simulink model "model"  (R2016a)
(part 2 of 3)

  _CN_201293312_500000_CN_216778426_500000 : powerlib/Elements/Distributed Parameters Line  Phases=3  Frequency=50  Resistance=[0.01273 0.3864]  Inductance="[0.9337e-3  4.1264e-3]"  Capacitance=[12.74e-9 7.751e-9]  Length=28.6125  x1=[8.73114913702011e-11 380000 380000;314.159265358979 314.159265358979 314.159265358979;-0.177670123217348 0.415246442777429 -1.15554988401747]  x2=[1.26090477118469e-09 381852.398472139 381852.398472139;314.159265358979 314.159265358979 314.159265358979;-1.41941675517191 0.415007521738739 -1.15578880505616]  x3=[1.07663708898761e-11 1405.24743813465 1405.24743813466;314.159265358979 314.159265358979 314.159265358979;-2.70558821102223 0.316110507002444 -1.25468581979246]  x4=[8.62234243168895e-12 1405.96374414071 1405.9637441407;314.159265358979 314.159265358979 314.159265358979;0.245769282942371 0.405640215255436 -1.16515611153945]  x5=0.000565541566995742  V1=ones(3,3)  V2=ones(3,3)  I1=ones(3,3)  I2=ones(3,3)  nHarmo=1  Measurements=None
  _CN_215451416_500000_CN215429864 : powerlib/Elements/Distributed Parameters Line  Phases=3  Frequency=50  Resistance=[0.01273 0.3864]  Inductance="[0.9337e-3  4.1264e-3]"  Capacitance=[12.74e-9 7.751e-9]  Length=72.2446  x1=[8.73114913702011e-11 380000 380000;314.159265358979 314.159265358979 314.159265358979;-0.177670123217348 0.415246442777429 -1.15554988401747]  x2=[1.26090477118469e-09 381852.398472139 381852.398472139;314.159265358979 314.159265358979 314.159265358979;-1.41941675517191 0.415007521738739 -1.15578880505616]  x3=[1.07663708898761e-11 1405.24743813465 1405.24743813466;314.159265358979 314.159265358979 314.159265358979;-2.70558821102223 0.316110507002444 -1.25468581979246]  x4=[8.62234243168895e-12 1405.96374414071 1405.9637441407;314.159265358979 314.159265358979 314.159265358979;0.245769282942371 0.405640215255436 -1.16515611153945]  x5=0.000565541566995742  V1=ones(3,3)  V2=ones(3,3)  I1=ones(3,3)  I2=ones(3,3)  nHarmo=1  Measurements=None
  _CN_232998815_275000_CN233174201 : powerlib/Elements/Distributed Parameters Line  Phases=3  Frequency=50  Resistance=[0.01273 0.3864]  Inductance="[0.9337e-3  4.1264e-3]"  Capacitance=[12.74e-9 7.751e-9]  Length=1.0529  x1=[8.73114913702011e-11 380000 380000;314.159265358979 314.159265358979 314.159265358979;-0.177670123217348 0.415246442777429 -1.15554988401747]  x2=[1.26090477118469e-09 381852.398472139 381852.398472139;314.159265358979 314.159265358979 314.159265358979;-1.41941675517191 0.415007521738739 -1.15578880505616]  x3=[1.07663708898761e-11 1405.24743813465 1405.24743813466;314.159265358979 314.159265358979 314.159265358979;-2.70558821102223 0.316110507002444 -1.25468581979246]  x4=[8.62234243168895e-12 1405.96374414071 1405.9637441407;314.159265358979 314.159265358979 314.159265358979;0.245769282942371 0.405640215255436 -1.16515611153945]  x5=0.000565541566995742  V1=ones(3,3)  V2=ones(3,3)  I1=ones(3,3)  I2=ones(3,3)  nHarmo=1  Measurements=None
  _CN_241828221_500000_CN_241822623_500000 : powerlib/Elements/Distributed Parameters Line  Phases=3  Frequency=50  Resistance=[0.01273 0.3864]  Inductance="[0.9337e-3  4.1264e-3]"  Capacitance=[12.74e-9 7.751e-9]  Length=76.1994  x1=[8.73114913702011e-11 380000 380000;314.159265358979 314.159265358979 314.159265358979;-0.177670123217348 0.415246442777429 -1.15554988401747]  x2=[1.26090477118469e-09 381852.398472139 381852.398472139;314.159265358979 314.159265358979 314.159265358979;-1.41941675517191 0.415007521738739 -1.15578880505616]  x3=[1.07663708898761e-11 1405.24743813465 1405.24743813466;314.159265358979 314.159265358979 314.159265358979;-2.70558821102223 0.316110507002444 -1.25468581979246]  x4=[8.62234243168895e-12 1405.96374414071 1405.9637441407;314.159265358979 314.159265358979 314.159265358979;0.245769282942371 0.405640215255436 -1.16515611153945]  x5=0.000565541566995742  V1=ones(3,3)  V2=ones(3,3)  I1=ones(3,3)  I2=ones(3,3)  nHarmo=1  Measurements=None
  _CN_241956440_275000_CN214992492 : powerlib/Elements/Distributed Parameters Line  Phases=3  Frequency=50  Resistance=[0.01273 0.3864]  Inductance="[0.9337e-3  4.1264e-3]"  Capacitance=[12.74e-9 7.751e-9]  Length=68.4368  x1=[8.73114913702011e-11 380000 380000;314.159265358979 314.159265358979 314.159265358979;-0.177670123217348 0.415246442777429 -1.15554988401747]  x2=[1.26090477118469e-09 381852.398472139 381852.398472139;314.159265358979 314.159265358979 314.159265358979;-1.41941675517191 0.415007521738739 -1.15578880505616]  x3=[1.07663708898761e-11 1405.24743813465 1405.24743813466;314.159265358979 314.159265358979 314.159265358979;-2.70558821102223 0.316110507002444 -1.25468581979246]  x4=[8.62234243168895e-12 1405.96374414071 1405.9637441407;314.159265358979 314.159265358979 314.159265358979;0.245769282942371 0.405640215255436 -1.16515611153945]  x5=0.000565541566995742  V1=ones(3,3)  V2=ones(3,3)  I1=ones(3,3)  I2=ones(3,3)  nHarmo=1  Measurements=None
  _CN_241956440_275000_CN_241923317_275000 : powerlib/Elements/Distributed Parameters Line  Phases=3  Frequency=50  Resistance=[0.01273 0.3864]  Inductance="[0.9337e-3  4.1264e-3]"  Capacitance=[12.74e-9 7.751e-9]  Length=27.3525  x1=[8.73114913702011e-11 380000 380000;314.159265358979 314.159265358979 314.159265358979;-0.177670123217348 0.415246442777429 -1.15554988401747]  x2=[1.26090477118469e-09 381852.398472139 381852.398472139;314.159265358979 314.159265358979 314.159265358979;-1.41941675517191 0.415007521738739 -1.15578880505616]  x3=[1.07663708898761e-11 1405.24743813465 1405.24743813466;314.159265358979 314.159265358979 314.159265358979;-2.70558821102223 0.316110507002444 -1.25468581979246]  x4=[8.62234243168895e-12 1405.96374414071 1405.9637441407;314.159265358979 314.159265358979 314.159265358979;0.245769282942371 0.405640215255436 -1.16515611153945]  x5=0.000565541566995742  V1=ones(3,3)  V2=ones(3,3)  I1=ones(3,3)  I2=ones(3,3)  nHarmo=1  Measurements=None
  _CN_241956440_275000_CN_242532736_275000 : powerlib/Elements/Distributed Parameters Line  Phases=3  Frequency=50  Resistance=[0.01273 0.3864]  Inductance="[0.9337e-3  4.1264e-3]"  Capacitance=[12.74e-9 7.751e-9]  Length=38.0576  x1=[8.73114913702011e-11 380000 380000;314.159265358979 314.159265358979 314.159265358979;-0.177670123217348 0.415246442777429 -1.15554988401747]  x2=[1.26090477118469e-09 381852.398472139 381852.398472139;314.159265358979 314.159265358979 314.159265358979;-1.41941675517191 0.415007521738739 -1.15578880505616]  x3=[1.07663708898761e-11 1405.24743813465 1405.24743813466;314.159265358979 314.159265358979 314.159265358979;-2.70558821102223 0.316110507002444 -1.25468581979246]  x4=[8.62234243168895e-12 1405.96374414071 1405.9637441407;314.159265358979 314.159265358979 314.159265358979;0.245769282942371 0.405640215255436 -1.16515611153945]  x5=0.000565541566995742  V1=ones(3,3)  V2=ones(3,3)  I1=ones(3,3)  I2=ones(3,3)  nHarmo=1  Measurements=None
  _CN_242103481_500000_CN_241828221_500000 : powerlib/Elements/Distributed Parameters Line  Phases=3  Frequency=50  Resistance=[0.01273 0.3864]  Inductance="[0.9337e-3  4.1264e-3]"  Capacitance=[12.74e-9 7.751e-9]  Length=71.051  x1=[8.73114913702011e-11 380000 380000;314.159265358979 314.159265358979 314.159265358979;-0.177670123217348 0.415246442777429 -1.15554988401747]  x2=[1.26090477118469e-09 381852.398472139 381852.398472139;314.159265358979 314.159265358979 314.159265358979;-1.41941675517191 0.415007521738739 -1.15578880505616]  x3=[1.07663708898761e-11 1405.24743813465 1405.24743813466;314.159265358979 314.159265358979 314.159265358979;-2.70558821102223 0.316110507002444 -1.25468581979246]  x4=[8.62234243168895e-12 1405.96374414071 1405.9637441407;314.159265358979 314.159265358979 314.159265358979;0.245769282942371 0.405640215255436 -1.16515611153945]  x5=0.000565541566995742  V1=ones(3,3)  V2=ones(3,3)  I1=ones(3,3)  I2=ones(3,3)  nHarmo=1  Measurements=None
  _CN_242103481_500000_CN_317416612_500000 : powerlib/Elements/Distributed Parameters Line  Phases=3  Frequency=50  Resistance=[0.01273 0.3864]  Inductance="[0.9337e-3  4.1264e-3]"  Capacitance=[12.74e-9 7.751e-9]  Length=86.3859  x1=[8.73114913702011e-11 380000 380000;314.159265358979 314.159265358979 314.159265358979;-0.177670123217348 0.415246442777429 -1.15554988401747]  x2=[1.26090477118469e-09 381852.398472139 381852.398472139;314.159265358979 314.159265358979 314.159265358979;-1.41941675517191 0.415007521738739 -1.15578880505616]  x3=[1.07663708898761e-11 1405.24743813465 1405.24743813466;314.159265358979 314.159265358979 314.159265358979;-2.70558821102223 0.316110507002444 -1.25468581979246]  x4=[8.62234243168895e-12 1405.96374414071 1405.9637441407;314.159265358979 314.159265358979 314.159265358979;0.245769282942371 0.405640215255436 -1.16515611153945]  x5=0.000565541566995742  V1=ones(3,3)  V2=ones(3,3)  I1=ones(3,3)  I2=ones(3,3)  nHarmo=1  Measurements=None
  _CN_242103481_500000_CN_317511904_500000 : powerlib/Elements/Distributed Parameters Line  Phases=3  Frequency=50  Resistance=[0.01273 0.3864]  Inductance="[0.9337e-3  4.1264e-3]"  Capacitance=[12.74e-9 7.751e-9]  Length=50.2566  x1=[8.73114913702011e-11 380000 380000;314.159265358979 314.159265358979 314.159265358979;-0.177670123217348 0.415246442777429 -1.15554988401747]  x2=[1.26090477118469e-09 381852.398472139 381852.398472139;314.159265358979 314.159265358979 314.159265358979;-1.41941675517191 0.415007521738739 -1.15578880505616]  x3=[1.07663708898761e-11 1405.24743813465 1405.24743813466;314.159265358979 314.159265358979 314.159265358979;-2.70558821102223 0.316110507002444 -1.25468581979246]  x4=[8.62234243168895e-12 1405.96374414071 1405.9637441407;314.159265358979 314.159265358979 314.159265358979;0.245769282942371 0.405640215255436 -1.16515611153945]  x5=0.000565541566995742  V1=ones(3,3)  V2=ones(3,3)  I1=ones(3,3)  I2=ones(3,3)  nHarmo=1  Measurements=None
  _CN_242103532_500000_CN_241822623_500000 : powerlib/Elements/Distributed Parameters Line  Phases=3  Frequency=50  Resistance=[0.01273 0.3864]  Inductance="[0.9337e-3  4.1264e-3]"  Capacitance=[12.74e-9 7.751e-9]  Length=4.2886  x1=[8.73114913702011e-11 380000 380000;314.159265358979 314.159265358979 314.159265358979;-0.177670123217348 0.415246442777429 -1.15554988401747]  x2=[1.26090477118469e-09 381852.398472139 381852.398472139;314.159265358979 314.159265358979 314.159265358979;-1.41941675517191 0.415007521738739 -1.15578880505616]  x3=[1.07663708898761e-11 1405.24743813465 1405.24743813466;314.159265358979 314.159265358979 314.159265358979;-2.70558821102223 0.316110507002444 -1.25468581979246]  x4=[8.62234243168895e-12 1405.96374414071 1405.9637441407;314.159265358979 314.159265358979 314.159265358979;0.245769282942371 0.405640215255436 -1.16515611153945]  x5=0.000565541566995742  V1=ones(3,3)  V2=ones(3,3)  I1=ones(3,3)  I2=ones(3,3)  nHarmo=1  Measurements=None
  _CN_242253497_275000_CN_185032690_275000 : powerlib/Elements/Distributed Parameters Line  Phases=3  Frequency=50  Resistance=[0.01273 0.3864]  Inductance="[0.9337e-3  4.1264e-3]"  Capacitance=[12.74e-9 7.751e-9]  Length=66.6304  x1=[8.73114913702011e-11 380000 380000;314.159265358979 314.159265358979 314.159265358979;-0.177670123217348 0.415246442777429 -1.15554988401747]  x2=[1.26090477118469e-09 381852.398472139 381852.398472139;314.159265358979 314.159265358979 314.159265358979;-1.41941675517191 0.415007521738739 -1.15578880505616]  x3=[1.07663708898761e-11 1405.24743813465 1405.24743813466;314.159265358979 314.159265358979 314.159265358979;-2.70558821102223 0.316110507002444 -1.25468581979246]  x4=[8.62234243168895e-12 1405.96374414071 1405.9637441407;314.159265358979 314.159265358979 314.159265358979;0.245769282942371 0.405640215255436 -1.16515611153945]  x5=0.000565541566995742  V1=ones(3,3)  V2=ones(3,3)  I1=ones(3,3)  I2=ones(3,3)  nHarmo=1  Measurements=None
  _CN_242253500_500000_CN_204258596_500000 : powerlib/Elements/Distributed Parameters Line  Phases=3  Frequency=50  Resistance=[0.01273 0.3864]  Inductance="[0.9337e-3  4.1264e-3]"  Capacitance=[12.74e-9 7.751e-9]  Length=93.4711  x1=[8.73114913702011e-11 380000 380000;314.159265358979 314.159265358979 314.159265358979;-0.177670123217348 0.415246442777429 -1.15554988401747]  x2=[1.26090477118469e-09 381852.398472139 381852.398472139;314.159265358979 314.159265358979 314.159265358979;-1.41941675517191 0.415007521738739 -1.15578880505616]  x3=[1.07663708898761e-11 1405.24743813465 1405.24743813466;314.159265358979 314.159265358979 314.159265358979;-2.70558821102223 0.316110507002444 -1.25468581979246]  x4=[8.62234243168895e-12 1405.96374414071 1405.9637441407;314.159265358979 314.159265358979 314.159265358979;0.245769282942371 0.405640215255436 -1.16515611153945]  x5=0.000565541566995742  V1=ones(3,3)  V2=ones(3,3)  I1=ones(3,3)  I2=ones(3,3)  nHarmo=1  Measurements=None
  _CN_250430935_275000_CN354115662 : powerlib/Elements/Distributed Parameters Line  Phases=3  Frequency=50  Resistance=[0.01273 0.3864]  Inductance="[0.9337e-3  4.1264e-3]"  Capacitance=[12.74e-9 7.751e-9]  Length=98.2855  x1=[8.73114913702011e-11 380000 380000;314.159265358979 314.159265358979 314.159265358979;-0.177670123217348 0.415246442777429 -1.15554988401747]  x2=[1.26090477118469e-09 381852.398472139 381852.398472139;314.159265358979 314.159265358979 314.159265358979;-1.41941675517191 0.415007521738739 -1.15578880505616]  x3=[1.07663708898761e-11 1405.24743813465 1405.24743813466;314.159265358979 314.159265358979 314.159265358979;-2.70558821102223 0.316110507002444 -1.25468581979246]  x4=[8.62234243168895e-12 1405.96374414071 1405.9637441407;314.159265358979 314.159265358979 314.159265358979;0.245769282942371 0.405640215255436 -1.16515611153945]  x5=0.000565541566995742  V1=ones(3,3)  V2=ones(3,3)  I1=ones(3,3)  I2=ones(3,3)  nHarmo=1  Measurements=None
  _CN_250430935_275000_CN_107262429_275000 : powerlib/Elements/Distributed Parameters Line  Phases=3  Frequency=50  Resistance=[0.01273 0.3864]  Inductance="[0.9337e-3  4.1264e-3]"  Capacitance=[12.74e-9 7.751e-9]  Length=49.0738  x1=[8.73114913702011e-11 380000 380000;314.159265358979 314.159265358979 314.159265358979;-0.177670123217348 0.415246442777429 -1.15554988401747]  x2=[1.26090477118469e-09 381852.398472139 381852.398472139;314.159265358979 314.159265358979 314.159265358979;-1.41941675517191 0.415007521738739 -1.15578880505616]  x3=[1.07663708898761e-11 1405.24743813465 1405.24743813466;314.159265358979 314.159265358979 314.159265358979;-2.70558821102223 0.316110507002444 -1.25468581979246]  x4=[8.62234243168895e-12 1405.96374414071 1405.9637441407;314.159265358979 314.159265358979 314.159265358979;0.245769282942371 0.405640215255436 -1.16515611153945]  x5=0.000565541566995742  V1=ones(3,3)  V2=ones(3,3)  I1=ones(3,3)  I2=ones(3,3)  nHarmo=1  Measurements=None
  _CN_302164679_275000_CN_316581637_275000 : powerlib/Elements/Distributed Parameters Line  Phases=3  Frequency=50  Resistance=[0.01273 0.3864]  Inductance="[0.9337e-3  4.1264e-3]"  Capacitance=[12.74e-9 7.751e-9]  Length=35.2995  x1=[8.73114913702011e-11 380000 380000;314.159265358979 314.159265358979 314.159265358979;-0.177670123217348 0.415246442777429 -1.15554988401747]  x2=[1.26090477118469e-09 381852.398472139 381852.398472139;314.159265358979 314.159265358979 314.159265358979;-1.41941675517191 0.415007521738739 -1.15578880505616]  x3=[1.07663708898761e-11 1405.24743813465 1405.24743813466;314.159265358979 314.159265358979 314.159265358979;-2.70558821102223 0.316110507002444 -1.25468581979246]  x4=[8.62234243168895e-12 1405.96374414071 1405.9637441407;314.159265358979 314.159265358979 314.159265358979;0.245769282942371 0.405640215255436 -1.16515611153945]  x5=0.000565541566995742  V1=ones(3,3)  V2=ones(3,3)  I1=ones(3,3)  I2=ones(3,3)  nHarmo=1  Measurements=None
  _CN_315461272_500000_CN_105298089_500000 : powerlib/Elements/Distributed Parameters Line  Phases=3  Frequency=50  Resistance=[0.01273 0.3864]  Inductance="[0.9337e-3  4.1264e-3]"  Capacitance=[12.74e-9 7.751e-9]  Length=97.8057  x1=[8.73114913702011e-11 380000 380000;314.159265358979 314.159265358979 314.159265358979;-0.177670123217348 0.415246442777429 -1.15554988401747]  x2=[1.26090477118469e-09 381852.398472139 381852.398472139;314.159265358979 314.159265358979 314.159265358979;-1.41941675517191 0.415007521738739 -1.15578880505616]  x3=[1.07663708898761e-11 1405.24743813465 1405.24743813466;314.159265358979 314.159265358979 314.159265358979;-2.70558821102223 0.316110507002444 -1.25468581979246]  x4=[8.62234243168895e-12 1405.96374414071 1405.9637441407;314.159265358979 314.159265358979 314.159265358979;0.245769282942371 0.405640215255436 -1.16515611153945]  x5=0.000565541566995742  V1=ones(3,3)  V2=ones(3,3)  I1=ones(3,3)  I2=ones(3,3)  nHarmo=1  Measurements=None
  _CN_315608215_500000_CN_169249243_500000 : powerlib/Elements/Distributed Parameters Line  Phases=3  Frequency=50  Resistance=[0.01273 0.3864]  Inductance="[0.9337e-3  4.1264e-3]"  Capacitance=[12.74e-9 7.751e-9]  Length=85.9807  x1=[8.73114913702011e-11 380000 380000;314.159265358979 314.159265358979 314.159265358979;-0.177670123217348 0.415246442777429 -1.15554988401747]  x2=[1.26090477118469e-09 381852.398472139 381852.398472139;314.159265358979 314.159265358979 314.159265358979;-1.41941675517191 0.415007521738739 -1.15578880505616]  x3=[1.07663708898761e-11 1405.24743813465 1405.24743813466;314.159265358979 314.159265358979 314.159265358979;-2.70558821102223 0.316110507002444 -1.25468581979246]  x4=[8.62234243168895e-12 1405.96374414071 1405.9637441407;314.159265358979 314.159265358979 314.159265358979;0.245769282942371 0.405640215255436 -1.16515611153945]  x5=0.000565541566995742  V1=ones(3,3)  V2=ones(3,3)  I1=ones(3,3)  I2=ones(3,3)  nHarmo=1  Measurements=None
  _CN_315608215_500000_CN_169249247_500000 : powerlib/Elements/Distributed Parameters Line  Phases=3  Frequency=50  Resistance=[0.01273 0.3864]  Inductance="[0.9337e-3  4.1264e-3]"  Capacitance=[12.74e-9 7.751e-9]  Length=76.4137  x1=[8.73114913702011e-11 380000 380000;314.159265358979 314.159265358979 314.159265358979;-0.177670123217348 0.415246442777429 -1.15554988401747]  x2=[1.26090477118469e-09 381852.398472139 381852.398472139;314.159265358979 314.159265358979 314.159265358979;-1.41941675517191 0.415007521738739 -1.15578880505616]  x3=[1.07663708898761e-11 1405.24743813465 1405.24743813466;314.159265358979 314.159265358979 314.159265358979;-2.70558821102223 0.316110507002444 -1.25468581979246]  x4=[8.62234243168895e-12 1405.96374414071 1405.9637441407;314.159265358979 314.159265358979 314.159265358979;0.245769282942371 0.405640215255436 -1.16515611153945]  x5=0.000565541566995742  V1=ones(3,3)  V2=ones(3,3)  I1=ones(3,3)  I2=ones(3,3)  nHarmo=1  Measurements=None
  _CN_315614776_275000_CN_315614783_275000 : powerlib/Elements/Distributed Parameters Line  Phases=3  Frequency=50  Resistance=[0.01273 0.3864]  Inductance="[0.9337e-3  4.1264e-3]"  Capacitance=[12.74e-9 7.751e-9]  Length=12.0528  x1=[8.73114913702011e-11 380000 380000;314.159265358979 314.159265358979 314.159265358979;-0.177670123217348 0.415246442777429 -1.15554988401747]  x2=[1.26090477118469e-09 381852.398472139 381852.398472139;314.159265358979 314.159265358979 314.159265358979;-1.41941675517191 0.415007521738739 -1.15578880505616]  x3=[1.07663708898761e-11 1405.24743813465 1405.24743813466;314.159265358979 314.159265358979 314.159265358979;-2.70558821102223 0.316110507002444 -1.25468581979246]  x4=[8.62234243168895e-12 1405.96374414071 1405.9637441407;314.159265358979 314.159265358979 314.159265358979;0.245769282942371 0.405640215255436 -1.16515611153945]  x5=0.000565541566995742  V1=ones(3,3)  V2=ones(3,3)  I1=ones(3,3)  I2=ones(3,3)  nHarmo=1  Measurements=None
  _CN_316459359_275000_CN_107262429_275000 : powerlib/Elements/Distributed Parameters Line  Phases=3  Frequency=50  Resistance=[0.01273 0.3864]  Inductance="[0.9337e-3  4.1264e-3]"  Capacitance=[12.74e-9 7.751e-9]  Length=29.441  x1=[8.73114913702011e-11 380000 380000;314.159265358979 314.159265358979 314.159265358979;-0.177670123217348 0.415246442777429 -1.15554988401747]  x2=[1.26090477118469e-09 381852.398472139 381852.398472139;314.159265358979 314.159265358979 314.159265358979;-1.41941675517191 0.415007521738739 -1.15578880505616]  x3=[1.07663708898761e-11 1405.24743813465 1405.24743813466;314.159265358979 314.159265358979 314.159265358979;-2.70558821102223 0.316110507002444 -1.25468581979246]  x4=[8.62234243168895e-12 1405.96374414071 1405.9637441407;314.159265358979 314.159265358979 314.159265358979;0.245769282942371 0.405640215255436 -1.16515611153945]  x5=0.000565541566995742  V1=ones(3,3)  V2=ones(3,3)  I1=ones(3,3)  I2=ones(3,3)  nHarmo=1  Measurements=None
  _CN_316566585_275000_CN_174636874_275000 : powerlib/Elements/Distributed Parameters Line  Phases=3  Frequency=50  Resistance=[0.01273 0.3864]  Inductance="[0.9337e-3  4.1264e-3]"  Capacitance=[12.74e-9 7.751e-9]  Length=36.4336  x1=[8.73114913702011e-11 380000 380000;314.159265358979 314.159265358979 314.159265358979;-0.177670123217348 0.415246442777429 -1.15554988401747]  x2=[1.26090477118469e-09 381852.398472139 381852.398472139;314.159265358979 314.159265358979 314.159265358979;-1.41941675517191 0.415007521738739 -1.15578880505616]  x3=[1.07663708898761e-11 1405.24743813465 1405.24743813466;314.159265358979 314.159265358979 314.159265358979;-2.70558821102223 0.316110507002444 -1.25468581979246]  x4=[8.62234243168895e-12 1405.96374414071 1405.9637441407;314.159265358979 314.159265358979 314.159265358979;0.245769282942371 0.405640215255436 -1.16515611153945]  x5=0.000565541566995742  V1=ones(3,3)  V2=ones(3,3)  I1=ones(3,3)  I2=ones(3,3)  nHarmo=1  Measurements=None
  _CN_316566588_275000_CN_174636874_275000 : powerlib/Elements/Distributed Parameters Line  Phases=3  Frequency=50  Resistance=[0.01273 0.3864]  Inductance="[0.9337e-3  4.1264e-3]"  Capacitance=[12.74e-9 7.751e-9]  Length=100.2417  x1=[8.73114913702011e-11 380000 380000;314.159265358979 314.159265358979 314.159265358979;-0.177670123217348 0.415246442777429 -1.15554988401747]  x2=[1.26090477118469e-09 381852.398472139 381852.398472139;314.159265358979 314.159265358979 314.159265358979;-1.41941675517191 0.415007521738739 -1.15578880505616]  x3=[1.07663708898761e-11 1405.24743813465 1405.24743813466;314.159265358979 314.159265358979 314.159265358979;-2.70558821102223 0.316110507002444 -1.25468581979246]  x4=[8.62234243168895e-12 1405.96374414071 1405.9637441407;314.159265358979 314.159265358979 314.159265358979;0.245769282942371 0.405640215255436 -1.16515611153945]  x5=0.000565541566995742  V1=ones(3,3)  V2=ones(3,3)  I1=ones(3,3)  I2=ones(3,3)  nHarmo=1  Measurements=None
  _CN_316566588_275000_CN_308348224_275000 : powerlib/Elements/Distributed Parameters Line  Phases=3  Frequency=50  Resistance=[0.01273 0.3864]  Inductance="[0.9337e-3  4.1264e-3]"  Capacitance=[12.74e-9 7.751e-9]  Length=168.728  x1=[8.73114913702011e-11 380000 380000;314.159265358979 314.159265358979 314.159265358979;-0.177670123217348 0.415246442777429 -1.15554988401747]  x2=[1.26090477118469e-09 381852.398472139 381852.398472139;314.159265358979 314.159265358979 314.159265358979;-1.41941675517191 0.415007521738739 -1.15578880505616]  x3=[1.07663708898761e-11 1405.24743813465 1405.24743813466;314.159265358979 314.159265358979 314.159265358979;-2.70558821102223 0.316110507002444 -1.25468581979246]  x4=[8.62234243168895e-12 1405.96374414071 1405.9637441407;314.159265358979 314.159265358979 314.159265358979;0.245769282942371 0.405640215255436 -1.16515611153945]  x5=0.000565541566995742  V1=ones(3,3)  V2=ones(3,3)  I1=ones(3,3)  I2=ones(3,3)  nHarmo=1  Measurements=None
  _CN_316566588_275000_CN_316581632_275000 : powerlib/Elements/Distributed Parameters Line  Phases=3  Frequency=50  Resistance=[0.01273 0.3864]  Inductance="[0.9337e-3  4.1264e-3]"  Capacitance=[12.74e-9 7.751e-9]  Length=2.0576  x1=[8.73114913702011e-11 380000 380000;314.159265358979 314.159265358979 314.159265358979;-0.177670123217348 0.415246442777429 -1.15554988401747]  x2=[1.26090477118469e-09 381852.398472139 381852.398472139;314.159265358979 314.159265358979 314.159265358979;-1.41941675517191 0.415007521738739 -1.15578880505616]  x3=[1.07663708898761e-11 1405.24743813465 1405.24743813466;314.159265358979 314.159265358979 314.159265358979;-2.70558821102223 0.316110507002444 -1.25468581979246]  x4=[8.62234243168895e-12 1405.96374414071 1405.9637441407;314.159265358979 314.159265358979 314.159265358979;0.245769282942371 0.405640215255436 -1.16515611153945]  x5=0.000565541566995742  V1=ones(3,3)  V2=ones(3,3)  I1=ones(3,3)  I2=ones(3,3)  nHarmo=1  Measurements=None
  _CN_317416612_500000_CN_204258596_500000 : powerlib/Elements/Distributed Parameters Line  Phases=3  Frequency=50  Resistance=[0.01273 0.3864]  Inductance="[0.9337e-3  4.1264e-3]"  Capacitance=[12.74e-9 7.751e-9]  Length=29.4625  x1=[8.73114913702011e-11 380000 380000;314.159265358979 314.159265358979 314.159265358979;-0.177670123217348 0.415246442777429 -1.15554988401747]  x2=[1.26090477118469e-09 381852.398472139 381852.398472139;314.159265358979 314.159265358979 314.159265358979;-1.41941675517191 0.415007521738739 -1.15578880505616]  x3=[1.07663708898761e-11 1405.24743813465 1405.24743813466;314.159265358979 314.159265358979 314.159265358979;-2.70558821102223 0.316110507002444 -1.25468581979246]  x4=[8.62234243168895e-12 1405.96374414071 1405.9637441407;314.159265358979 314.159265358979 314.159265358979;0.245769282942371 0.405640215255436 -1.16515611153945]  x5=0.000565541566995742  V1=ones(3,3)  V2=ones(3,3)  I1=ones(3,3)  I2=ones(3,3)  nHarmo=1  Measurements=None
  _CN_318218831_275000_CN_169993955_275000 : powerlib/Elements/Distributed Parameters Line  Phases=3  Frequency=50  Resistance=[0.01273 0.3864]  Inductance="[0.9337e-3  4.1264e-3]"  Capacitance=[12.74e-9 7.751e-9]  Length=37.4693  x1=[8.73114913702011e-11 380000 380000;314.159265358979 314.159265358979 314.159265358979;-0.177670123217348 0.415246442777429 -1.15554988401747]  x2=[1.26090477118469e-09 381852.398472139 381852.398472139;314.159265358979 314.159265358979 314.159265358979;-1.41941675517191 0.415007521738739 -1.15578880505616]  x3=[1.07663708898761e-11 1405.24743813465 1405.24743813466;314.159265358979 314.159265358979 314.159265358979;-2.70558821102223 0.316110507002444 -1.25468581979246]  x4=[8.62234243168895e-12 1405.96374414071 1405.9637441407;314.159265358979 314.159265358979 314.159265358979;0.245769282942371 0.405640215255436 -1.16515611153945]  x5=0.000565541566995742  V1=ones(3,3)  V2=ones(3,3)  I1=ones(3,3)  I2=ones(3,3)  nHarmo=1  Measurements=None
  _CN_318218831_275000_CN_170016148_275000 : powerlib/Elements/Distributed Parameters Line  Phases=3  Frequency=50  Resistance=[0.01273 0.3864]  Inductance="[0.9337e-3  4.1264e-3]"  Capacitance=[12.74e-9 7.751e-9]  Length=35.0104  x1=[8.73114913702011e-11 380000 380000;314.159265358979 314.159265358979 314.159265358979;-0.177670123217348 0.415246442777429 -1.15554988401747]  x2=[1.26090477118469e-09 381852.398472139 381852.398472139;314.159265358979 314.159265358979 314.159265358979;-1.41941675517191 0.415007521738739 -1.15578880505616]  x3=[1.07663708898761e-11 1405.24743813465 1405.24743813466;314.159265358979 314.159265358979 314.159265358979;-2.70558821102223 0.316110507002444 -1.25468581979246]  x4=[8.62234243168895e-12 1405.96374414071 1405.9637441407;314.159265358979 314.159265358979 314.159265358979;0.245769282942371 0.405640215255436 -1.16515611153945]  x5=0.000565541566995742  V1=ones(3,3)  V2=ones(3,3)  I1=ones(3,3)  I2=ones(3,3)  nHarmo=1  Measurements=None
  _CN_318218831_275000_CN_319300956_275000 : powerlib/Elements/Distributed Parameters Line  Phases=3  Frequency=50  Resistance=[0.01273 0.3864]  Inductance="[0.9337e-3  4.1264e-3]"  Capacitance=[12.74e-9 7.751e-9]  Length=85.9941  x1=[8.73114913702011e-11 380000 380000;314.159265358979 314.159265358979 314.159265358979;-0.177670123217348 0.415246442777429 -1.15554988401747]  x2=[1.26090477118469e-09 381852.398472139 381852.398472139;314.159265358979 314.159265358979 314.159265358979;-1.41941675517191 0.415007521738739 -1.15578880505616]  x3=[1.07663708898761e-11 1405.24743813465 1405.24743813466;314.159265358979 314.159265358979 314.159265358979;-2.70558821102223 0.316110507002444 -1.25468581979246]  x4=[8.62234243168895e-12 1405.96374414071 1405.9637441407;314.159265358979 314.159265358979 314.159265358979;0.245769282942371 0.405640215255436 -1.16515611153945]  x5=0.000565541566995742  V1=ones(3,3)  V2=ones(3,3)  I1=ones(3,3)  I2=ones(3,3)  nHarmo=1  Measurements=None
  _CN_318302348_275000_CN319098734 : powerlib/Elements/Distributed Parameters Line  Phases=3  Frequency=50  Resistance=[0.01273 0.3864]  Inductance="[0.9337e-3  4.1264e-3]"  Capacitance=[12.74e-9 7.751e-9]  Length=47.29  x1=[8.73114913702011e-11 380000 380000;314.159265358979 314.159265358979 314.159265358979;-0.177670123217348 0.415246442777429 -1.15554988401747]  x2=[1.26090477118469e-09 381852.398472139 381852.398472139;314.159265358979 314.159265358979 314.159265358979;-1.41941675517191 0.415007521738739 -1.15578880505616]  x3=[1.07663708898761e-11 1405.24743813465 1405.24743813466;314.159265358979 314.159265358979 314.159265358979;-2.70558821102223 0.316110507002444 -1.25468581979246]  x4=[8.62234243168895e-12 1405.96374414071 1405.9637441407;314.159265358979 314.159265358979 314.159265358979;0.245769282942371 0.405640215255436 -1.16515611153945]  x5=0.000565541566995742  V1=ones(3,3)  V2=ones(3,3)  I1=ones(3,3)  I2=ones(3,3)  nHarmo=1  Measurements=None
  _CN_320438391_500000_CN_110682956_500000 : powerlib/Elements/Distributed Parameters Line  Phases=3  Frequency=50  Resistance=[0.01273 0.3864]  Inductance="[0.9337e-3  4.1264e-3]"  Capacitance=[12.74e-9 7.751e-9]  Length=125.4052  x1=[8.73114913702011e-11 380000 380000;314.159265358979 314.159265358979 314.159265358979;-0.177670123217348 0.415246442777429 -1.15554988401747]  x2=[1.26090477118469e-09 381852.398472139 381852.398472139;314.159265358979 314.159265358979 314.159265358979;-1.41941675517191 0.415007521738739 -1.15578880505616]  x3=[1.07663708898761e-11 1405.24743813465 1405.24743813466;314.159265358979 314.159265358979 314.159265358979;-2.70558821102223 0.316110507002444 -1.25468581979246]  x4=[8.62234243168895e-12 1405.96374414071 1405.9637441407;314.159265358979 314.159265358979 314.159265358979;0.245769282942371 0.405640215255436 -1.16515611153945]  x5=0.000565541566995742  V1=ones(3,3)  V2=ones(3,3)  I1=ones(3,3)  I2=ones(3,3)  nHarmo=1  Measurements=None
  _CN_320438391_500000_CN_169031921_500000 : powerlib/Elements/Distributed Parameters Line  Phases=3  Frequency=50  Resistance=[0.01273 0.3864]  Inductance="[0.9337e-3  4.1264e-3]"  Capacitance=[12.74e-9 7.751e-9]  Length=17.5679  x1=[8.73114913702011e-11 380000 380000;314.159265358979 314.159265358979 314.159265358979;-0.177670123217348 0.415246442777429 -1.15554988401747]  x2=[1.26090477118469e-09 381852.398472139 381852.398472139;314.159265358979 314.159265358979 314.159265358979;-1.41941675517191 0.415007521738739 -1.15578880505616]  x3=[1.07663708898761e-11 1405.24743813465 1405.24743813466;314.159265358979 314.159265358979 314.159265358979;-2.70558821102223 0.316110507002444 -1.25468581979246]  x4=[8.62234243168895e-12 1405.96374414071 1405.9637441407;314.159265358979 314.159265358979 314.159265358979;0.245769282942371 0.405640215255436 -1.16515611153945]  x5=0.000565541566995742  V1=ones(3,3)  V2=ones(3,3)  I1=ones(3,3)  I2=ones(3,3)  nHarmo=1  Measurements=None
  _CN_320438391_500000_CN_241822621_500000 : powerlib/Elements/Distributed Parameters Line  Phases=3  Frequency=50  Resistance=[0.01273 0.3864]  Inductance="[0.9337e-3  4.1264e-3]"  Capacitance=[12.74e-9 7.751e-9]  Length=111.5076  x1=[8.73114913702011e-11 380000 380000;314.159265358979 314.159265358979 314.159265358979;-0.177670123217348 0.415246442777429 -1.15554988401747]  x2=[1.26090477118469e-09 381852.398472139 381852.398472139;314.159265358979 314.159265358979 314.159265358979;-1.41941675517191 0.415007521738739 -1.15578880505616]  x3=[1.07663708898761e-11 1405.24743813465 1405.24743813466;314.159265358979 314.159265358979 314.159265358979;-2.70558821102223 0.316110507002444 -1.25468581979246]  x4=[8.62234243168895e-12 1405.96374414071 1405.9637441407;314.159265358979 314.159265358979 314.159265358979;0.245769282942371 0.405640215255436 -1.16515611153945]  x5=0.000565541566995742  V1=ones(3,3)  V2=ones(3,3)  I1=ones(3,3)  I2=ones(3,3)  nHarmo=1  Measurements=None
  _CN_320438391_500000_CN_320444665_500000 : powerlib/Elements/Distributed Parameters Line  Phases=3  Frequency=50  Resistance=[0.01273 0.3864]  Inductance="[0.9337e-3  4.1264e-3]"  Capacitance=[12.74e-9 7.751e-9]  Length=72.722  x1=[8.73114913702011e-11 380000 380000;314.159265358979 314.159265358979 314.159265358979;-0.177670123217348 0.415246442777429 -1.15554988401747]  x2=[1.26090477118469e-09 381852.398472139 381852.398472139;314.159265358979 314.159265358979 314.159265358979;-1.41941675517191 0.415007521738739 -1.15578880505616]  x3=[1.07663708898761e-11 1405.24743813465 1405.24743813466;314.159265358979 314.159265358979 314.159265358979;-2.70558821102223 0.316110507002444 -1.25468581979246]  x4=[8.62234243168895e-12 1405.96374414071 1405.9637441407;314.159265358979 314.159265358979 314.159265358979;0.245769282942371 0.405640215255436 -1.16515611153945]  x5=0.000565541566995742  V1=ones(3,3)  V2=ones(3,3)  I1=ones(3,3)  I2=ones(3,3)  nHarmo=1  Measurements=None
  _CN_325868333_275000_CN_110682951_275000 : powerlib/Elements/Distributed Parameters Line  Phases=3  Frequency=50  Resistance=[0.01273 0.3864]  Inductance="[0.9337e-3  4.1264e-3]"  Capacitance=[12.74e-9 7.751e-9]  Length=59.702  x1=[8.73114913702011e-11 380000 380000;314.159265358979 314.159265358979 314.159265358979;-0.177670123217348 0.415246442777429 -1.15554988401747]  x2=[1.26090477118469e-09 381852.398472139 381852.398472139;314.159265358979 314.159265358979 314.159265358979;-1.41941675517191 0.415007521738739 -1.15578880505616]  x3=[1.07663708898761e-11 1405.24743813465 1405.24743813466;314.159265358979 314.159265358979 314.159265358979;-2.70558821102223 0.316110507002444 -1.25468581979246]  x4=[8.62234243168895e-12 1405.96374414071 1405.9637441407;314.159265358979 314.159265358979 314.159265358979;0.245769282942371 0.405640215255436 -1.16515611153945]  x5=0.000565541566995742  V1=ones(3,3)  V2=ones(3,3)  I1=ones(3,3)  I2=ones(3,3)  nHarmo=1  Measurements=None
  _CN_66098469_500000_CN216480979 : powerlib/Elements/Distributed Parameters Line  Phases=3  Frequency=50  Resistance=[0.01273 0.3864]  Inductance="[0.9337e-3  4.1264e-3]"  Capacitance=[12.74e-9 7.751e-9]  Length=100.2  x1=[8.73114913702011e-11 380000 380000;314.159265358979 314.159265358979 314.159265358979;-0.177670123217348 0.415246442777429 -1.15554988401747]  x2=[1.26090477118469e-09 381852.398472139 381852.398472139;314.159265358979 314.159265358979 314.159265358979;-1.41941675517191 0.415007521738739 -1.15578880505616]  x3=[1.07663708898761e-11 1405.24743813465 1405.24743813466;314.159265358979 314.159265358979 314.159265358979;-2.70558821102223 0.316110507002444 -1.25468581979246]  x4=[8.62234243168895e-12 1405.96374414071 1405.9637441407;314.159265358979 314.159265358979 314.159265358979;0.245769282942371 0.405640215255436 -1.16515611153945]  x5=0.000565541566995742  V1=ones(3,3)  V2=ones(3,3)  I1=ones(3,3)  I2=ones(3,3)  nHarmo=1  Measurements=None
  _CN_87538349_500000_CN_102958903_500000 : powerlib/Elements/Distributed Parameters Line  Phases=3  Frequency=50  Resistance=[0.01273 0.3864]  Inductance="[0.9337e-3  4.1264e-3]"  Capacitance=[12.74e-9 7.751e-9]  Length=23.1253  x1=[8.73114913702011e-11 380000 380000;314.159265358979 314.159265358979 314.159265358979;-0.177670123217348 0.415246442777429 -1.15554988401747]  x2=[1.26090477118469e-09 381852.398472139 381852.398472139;314.159265358979 314.159265358979 314.159265358979;-1.41941675517191 0.415007521738739 -1.15578880505616]  x3=[1.07663708898761e-11 1405.24743813465 1405.24743813466;314.159265358979 314.159265358979 314.159265358979;-2.70558821102223 0.316110507002444 -1.25468581979246]  x4=[8.62234243168895e-12 1405.96374414071 1405.9637441407;314.159265358979 314.159265358979 314.159265358979;0.245769282942371 0.405640215255436 -1.16515611153945]  x5=0.000565541566995742  V1=ones(3,3)  V2=ones(3,3)  I1=ones(3,3)  I2=ones(3,3)  nHarmo=1  Measurements=None
  _CN_87538349_500000_CN_171066843_500000 : powerlib/Elements/Distributed Parameters Line  Phases=3  Frequency=50  Resistance=[0.01273 0.3864]  Inductance="[0.9337e-3  4.1264e-3]"  Capacitance=[12.74e-9 7.751e-9]  Length=75.601  x1=[8.73114913702011e-11 380000 380000;314.159265358979 314.159265358979 314.159265358979;-0.177670123217348 0.415246442777429 -1.15554988401747]  x2=[1.26090477118469e-09 381852.398472139 381852.398472139;314.159265358979 314.159265358979 314.159265358979;-1.41941675517191 0.415007521738739 -1.15578880505616]  x3=[1.07663708898761e-11 1405.24743813465 1405.24743813466;314.159265358979 314.159265358979 314.159265358979;-2.70558821102223 0.316110507002444 -1.25468581979246]  x4=[8.62234243168895e-12 1405.96374414071 1405.9637441407;314.159265358979 314.159265358979 314.159265358979;0.245769282942371 0.405640215255436 -1.16515611153945]  x5=0.000565541566995742  V1=ones(3,3)  V2=ones(3,3)  I1=ones(3,3)  I2=ones(3,3)  nHarmo=1  Measurements=None
  _CN_87682157_275000_CN_128581912_275000 : powerlib/Elements/Distributed Parameters Line  Phases=3  Frequency=50  Resistance=[0.01273 0.3864]  Inductance="[0.9337e-3  4.1264e-3]"  Capacitance=[12.74e-9 7.751e-9]  Length=10.5143  x1=[8.73114913702011e-11 380000 380000;314.159265358979 314.159265358979 314.159265358979;-0.177670123217348 0.415246442777429 -1.15554988401747]  x2=[1.26090477118469e-09 381852.398472139 381852.398472139;314.159265358979 314.159265358979 314.159265358979;-1.41941675517191 0.415007521738739 -1.15578880505616]  x3=[1.07663708898761e-11 1405.24743813465 1405.24743813466;314.159265358979 314.159265358979 314.159265358979;-2.70558821102223 0.316110507002444 -1.25468581979246]  x4=[8.62234243168895e-12 1405.96374414071 1405.9637441407;314.159265358979 314.159265358979 314.159265358979;0.245769282942371 0.405640215255436 -1.16515611153945]  x5=0.000565541566995742  V1=ones(3,3)  V2=ones(3,3)  I1=ones(3,3)  I2=ones(3,3)  nHarmo=1  Measurements=None
  _CN_87682157_275000_CN_159491797_275000 : powerlib/Elements/Distributed Parameters Line  Phases=3  Frequency=50  Resistance=[0.01273 0.3864]  Inductance="[0.9337e-3  4.1264e-3]"  Capacitance=[12.74e-9 7.751e-9]  Length=8.1791  x1=[8.73114913702011e-11 380000 380000;314.159265358979 314.159265358979 314.159265358979;-0.177670123217348 0.415246442777429 -1.15554988401747]  x2=[1.26090477118469e-09 381852.398472139 381852.398472139;314.159265358979 314.159265358979 314.159265358979;-1.41941675517191 0.415007521738739 -1.15578880505616]  x3=[1.07663708898761e-11 1405.24743813465 1405.24743813466;314.159265358979 314.159265358979 314.159265358979;-2.70558821102223 0.316110507002444 -1.25468581979246]  x4=[8.62234243168895e-12 1405.96374414071 1405.9637441407;314.159265358979 314.159265358979 314.159265358979;0.245769282942371 0.405640215255436 -1.16515611153945]  x5=0.000565541566995742  V1=ones(3,3)  V2=ones(3,3)  I1=ones(3,3)  I2=ones(3,3)  nHarmo=1  Measurements=None
  powergui : powerlib/powergui  Priority=1  SimulationMode=Phasor  SolverType=Tustin/Backward Euler (TBE)  SampleTime=50e-6  frequency=50  SPID=off  DisableSnubberDevices=off  DisableRonSwitches=off  DisableVfSwitches=off  SwTol=0  DisplayEquations=off  Interpol=off  ExternalGateDelay=off  methode=off  Ts=10  FunctionMessages=off  echomessages=off  HookPort=off  EnableUseOfTLC=off  x0status=blocks  frequencyindice=50  Pbase=3000e6  ErrMax=0.0001  Iterations=50  UnitsV=V  UnitsW=W  buscounter=0  RestoreLinks=warning  ResistiveCurrentMeasurement=off  Frange=[0:2:500]  Ylog=off  Xlog=on  ShowGrid=off  save=off  variable=ZData  structure=0  ZoomFFT=off  StartTime=0.0  cycles=1  DisplayStyle=1  fundamental=60  FreqAxis=off  MaxFrequency=1000  frequencyindicesteady=1  RmsSteady=1  display=off
  丸山幹線_(Maruyama_Kansen)_CN_192745005_275000_CN_161946848_275000 : powerlib/Elements/Distributed Parameters Line  Phases=3  Frequency=50  Resistance=[0.01273 0.3864]  Inductance="[0.9337e-3  4.1264e-3]"  Capacitance=[12.74e-9 7.751e-9]  Length=36.5721  x1=[8.73114913702011e-11 380000 380000;314.159265358979 314.159265358979 314.159265358979;-0.177670123217348 0.415246442777429 -1.15554988401747]  x2=[1.26090477118469e-09 381852.398472139 381852.398472139;314.159265358979 314.159265358979 314.159265358979;-1.41941675517191 0.415007521738739 -1.15578880505616]  x3=[1.07663708898761e-11 1405.24743813465 1405.24743813466;314.159265358979 314.159265358979 314.159265358979;-2.70558821102223 0.316110507002444 -1.25468581979246]  x4=[8.62234243168895e-12 1405.96374414071 1405.9637441407;314.159265358979 314.159265358979 314.159265358979;0.245769282942371 0.405640215255436 -1.16515611153945]  x5=0.000565541566995742  V1=ones(3,3)  V2=ones(3,3)  I1=ones(3,3)  I2=ones(3,3)  nHarmo=1  Measurements=None
  京浜線1;2号線_CN_128364781_275000_CN_47110637_275000 : powerlib/Elements/Distributed Parameters Line  Phases=3  Frequency=50  Resistance=[0.01273 0.3864]  Inductance="[0.9337e-3  4.1264e-3]"  Capacitance=[12.74e-9 7.751e-9]  Length=27.5466  x1=[8.73114913702011e-11 380000 380000;314.159265358979 314.159265358979 314.159265358979;-0.177670123217348 0.415246442777429 -1.15554988401747]  x2=[1.26090477118469e-09 381852.398472139 381852.398472139;314.159265358979 314.159265358979 314.159265358979;-1.41941675517191 0.415007521738739 -1.15578880505616]  x3=[1.07663708898761e-11 1405.24743813465 1405.24743813466;314.159265358979 314.159265358979 314.159265358979;-2.70558821102223 0.316110507002444 -1.25468581979246]  x4=[8.62234243168895e-12 1405.96374414071 1405.9637441407;314.159265358979 314.159265358979 314.159265358979;0.245769282942371 0.405640215255436 -1.16515611153945]  x5=0.000565541566995742  V1=ones(3,3)  V2=ones(3,3)  I1=ones(3,3)  I2=ones(3,3)  nHarmo=1  Measurements=None
  伊勢幹線_CN_241956440_275000_CN_170793703_275000 : powerlib/Elements/Distributed Parameters Line  Phases=3  Frequency=50  Resistance=[0.01273 0.3864]  Inductance="[0.9337e-3  4.1264e-3]"  Capacitance=[12.74e-9 7.751e-9]  Length=139.4529  x1=[8.73114913702011e-11 380000 380000;314.159265358979 314.159265358979 314.159265358979;-0.177670123217348 0.415246442777429 -1.15554988401747]  x2=[1.26090477118469e-09 381852.398472139 381852.398472139;314.159265358979 314.159265358979 314.159265358979;-1.41941675517191 0.415007521738739 -1.15578880505616]  x3=[1.07663708898761e-11 1405.24743813465 1405.24743813466;314.159265358979 314.159265358979 314.159265358979;-2.70558821102223 0.316110507002444 -1.25468581979246]  x4=[8.62234243168895e-12 1405.96374414071 1405.9637441407;314.159265358979 314.159265358979 314.159265358979;0.245769282942371 0.405640215255436 -1.16515611153945]  x5=0.000565541566995742  V1=ones(3,3)  V2=ones(3,3)  I1=ones(3,3)  I2=ones(3,3)  nHarmo=1  Measurements=None
  佐久間東幹線_CN_116828675_275000_CN134376414 : powerlib/Elements/Distributed Parameters Line  Phases=3  Frequency=50  Resistance=[0.01273 0.3864]  Inductance="[0.9337e-3  4.1264e-3]"  Capacitance=[12.74e-9 7.751e-9]  Length=211.2094  x1=[8.73114913702011e-11 380000 380000;314.159265358979 314.159265358979 314.159265358979;-0.177670123217348 0.415246442777429 -1.15554988401747]  x2=[1.26090477118469e-09 381852.398472139 381852.398472139;314.159265358979 314.159265358979 314.159265358979;-1.41941675517191 0.415007521738739 -1.15578880505616]  x3=[1.07663708898761e-11 1405.24743813465 1405.24743813466;314.159265358979 314.159265358979 314.159265358979;-2.70558821102223 0.316110507002444 -1.25468581979246]  x4=[8.62234243168895e-12 1405.96374414071 1405.9637441407;314.159265358979 314.159265358979 314.159265358979;0.245769282942371 0.405640215255436 -1.16515611153945]  x5=0.000565541566995742  V1=ones(3,3)  V2=ones(3,3)  I1=ones(3,3)  I2=ones(3,3)  nHarmo=1  Measurements=None
  信濃幹線_CN_209726348_500000_CN_209429410_500000 : powerlib/Elements/Distributed Parameters Line  Phases=3  Frequency=50  Resistance=[0.01273 0.3864]  Inductance="[0.9337e-3  4.1264e-3]"  Capacitance=[12.74e-9 7.751e-9]  Length=54.9455  x1=[8.73114913702011e-11 380000 380000;314.159265358979 314.159265358979 314.159265358979;-0.177670123217348 0.415246442777429 -1.15554988401747]  x2=[1.26090477118469e-09 381852.398472139 381852.398472139;314.159265358979 314.159265358979 314.159265358979;-1.41941675517191 0.415007521738739 -1.15578880505616]  x3=[1.07663708898761e-11 1405.24743813465 1405.24743813466;314.159265358979 314.159265358979 314.159265358979;-2.70558821102223 0.316110507002444 -1.25468581979246]  x4=[8.62234243168895e-12 1405.96374414071 1405.9637441407;314.159265358979 314.159265358979 314.159265358979;0.245769282942371 0.405640215255436 -1.16515611153945]  x5=0.000565541566995742  V1=ones(3,3)  V2=ones(3,3)  I1=ones(3,3)  I2=ones(3,3)  nHarmo=1  Measurements=None
  加賀福光線_CN_169249243_500000_CN_169249247_500000 : powerlib/Elements/Distributed Parameters Line  Phases=3  Frequency=50  Resistance=[0.01273 0.3864]  Inductance="[0.9337e-3  4.1264e-3]"  Capacitance=[12.74e-9 7.751e-9]  Length=15.9777  x1=[8.73114913702011e-11 380000 380000;314.159265358979 314.159265358979 314.159265358979;-0.177670123217348 0.415246442777429 -1.15554988401747]  x2=[1.26090477118469e-09 381852.398472139 381852.398472139;314.159265358979 314.159265358979 314.159265358979;-1.41941675517191 0.415007521738739 -1.15578880505616]  x3=[1.07663708898761e-11 1405.24743813465 1405.24743813466;314.159265358979 314.159265358979 314.159265358979;-2.70558821102223 0.316110507002444 -1.25468581979246]  x4=[8.62234243168895e-12 1405.96374414071 1405.9637441407;314.159265358979 314.159265358979 314.159265358979;0.245769282942371 0.405640215255436 -1.16515611153945]  x5=0.000565541566995742  V1=ones(3,3)  V2=ones(3,3)  I1=ones(3,3)  I2=ones(3,3)  nHarmo=1  Measurements=None
  北葛城線_(Kita_Katsuragi_Sen)_CN_160374974_275000_CN_109834508_275000 : powerlib/Elements/Distributed Parameters Line  Phases=3  Frequency=50  Resistance=[0.01273 0.3864]  Inductance="[0.9337e-3  4.1264e-3]"  Capacitance=[12.74e-9 7.751e-9]  Length=23.6213  x1=[8.73114913702011e-11 380000 380000;314.159265358979 314.159265358979 314.159265358979;-0.177670123217348 0.415246442777429 -1.15554988401747]  x2=[1.26090477118469e-09 381852.398472139 381852.398472139;314.159265358979 314.159265358979 314.159265358979;-1.41941675517191 0.415007521738739 -1.15578880505616]  x3=[1.07663708898761e-11 1405.24743813465 1405.24743813466;314.159265358979 314.159265358979 314.159265358979;-2.70558821102223 0.316110507002444 -1.25468581979246]  x4=[8.62234243168895e-12 1405.96374414071 1405.9637441407;314.159265358979 314.159265358979 314.159265358979;0.245769282942371 0.405640215255436 -1.16515611153945]  x5=0.000565541566995742  V1=ones(3,3)  V2=ones(3,3)  I1=ones(3,3)  I2=ones(3,3)  nHarmo=1  Measurements=None
  南信幹線_CN_209429410_500000_CN_142662111_500000 : powerlib/Elements/Distributed Parameters Line  Phases=3  Frequency=50  Resistance=[0.01273 0.3864]  Inductance="[0.9337e-3  4.1264e-3]"  Capacitance=[12.74e-9 7.751e-9]  Length=85.8933  x1=[8.73114913702011e-11 380000 380000;314.159265358979 314.159265358979 314.159265358979;-0.177670123217348 0.415246442777429 -1.15554988401747]  x2=[1.26090477118469e-09 381852.398472139 381852.398472139;314.159265358979 314.159265358979 314.159265358979;-1.41941675517191 0.415007521738739 -1.15578880505616]  x3=[1.07663708898761e-11 1405.24743813465 1405.24743813466;314.159265358979 314.159265358979 314.159265358979;-2.70558821102223 0.316110507002444 -1.25468581979246]  x4=[8.62234243168895e-12 1405.96374414071 1405.9637441407;314.159265358979 314.159265358979 314.159265358979;0.245769282942371 0.405640215255436 -1.16515611153945]  x5=0.000565541566995742  V1=ones(3,3)  V2=ones(3,3)  I1=ones(3,3)  I2=ones(3,3)  nHarmo=1  Measurements=None
  富津火力線_CN_315461259_500000_CN_315461272_500000 : powerlib/Elements/Distributed Parameters Line  Phases=3  Frequency=50  Resistance=[0.01273 0.3864]  Inductance="[0.9337e-3  4.1264e-3]"  Capacitance=[12.74e-9 7.751e-9]  Length=36.2426  x1=[8.73114913702011e-11 380000 380000;314.159265358979 314.159265358979 314.159265358979;-0.177670123217348 0.415246442777429 -1.15554988401747]  x2=[1.26090477118469e-09 381852.398472139 381852.398472139;314.159265358979 314.159265358979 314.159265358979;-1.41941675517191 0.415007521738739 -1.15578880505616]  x3=[1.07663708898761e-11 1405.24743813465 1405.24743813466;314.159265358979 314.159265358979 314.159265358979;-2.70558821102223 0.316110507002444 -1.25468581979246]  x4=[8.62234243168895e-12 1405.96374414071 1405.9637441407;314.159265358979 314.159265358979 314.159265358979;0.245769282942371 0.405640215255436 -1.16515611153945]  x5=0.000565541566995742  V1=ones(3,3)  V2=ones(3,3)  I1=ones(3,3)  I2=ones(3,3)  nHarmo=1  Measurements=None
  小丸川幹線_CN_216956620_500000_CN216953915 : powerlib/Elements/Distributed Parameters Line  Phases=3  Frequency=50  Resistance=[0.01273 0.3864]  Inductance="[0.9337e-3  4.1264e-3]"  Capacitance=[12.74e-9 7.751e-9]  Length=54.7033  x1=[8.73114913702011e-11 380000 380000;314.159265358979 314.159265358979 314.159265358979;-0.177670123217348 0.415246442777429 -1.15554988401747]  x2=[1.26090477118469e-09 381852.398472139 381852.398472139;314.159265358979 314.159265358979 314.159265358979;-1.41941675517191 0.415007521738739 -1.15578880505616]  x3=[1.07663708898761e-11 1405.24743813465 1405.24743813466;314.159265358979 314.159265358979 314.159265358979;-2.70558821102223 0.316110507002444 -1.25468581979246]  x4=[8.62234243168895e-12 1405.96374414071 1405.9637441407;314.159265358979 314.159265358979 314.159265358979;0.245769282942371 0.405640215255436 -1.16515611153945]  x5=0.000565541566995742  V1=ones(3,3)  V2=ones(3,3)  I1=ones(3,3)  I2=ones(3,3)  nHarmo=1  Measurements=None
  志賀中能登線_CN_315608215_500000_CN255763556 : powerlib/Elements/Distributed Parameters Line  Phases=3  Frequency=50  Resistance=[0.01273 0.3864]  Inductance="[0.9337e-3  4.1264e-3]"  Capacitance=[12.74e-9 7.751e-9]  Length=19.0019  x1=[8.73114913702011e-11 380000 380000;314.159265358979 314.159265358979 314.159265358979;-0.177670123217348 0.415246442777429 -1.15554988401747]  x2=[1.26090477118469e-09 381852.398472139 381852.398472139;314.159265358979 314.159265358979 314.159265358979;-1.41941675517191 0.415007521738739 -1.15578880505616]  x3=[1.07663708898761e-11 1405.24743813465 1405.24743813466;314.159265358979 314.159265358979 314.159265358979;-2.70558821102223 0.316110507002444 -1.25468581979246]  x4=[8.62234243168895e-12 1405.96374414071 1405.9637441407;314.159265358979 314.159265358979 314.159265358979;0.245769282942371 0.405640215255436 -1.16515611153945]  x5=0.000565541566995742  V1=ones(3,3)  V2=ones(3,3)  I1=ones(3,3)  I2=ones(3,3)  nHarmo=1  Measurements=None
  房総線_CN_151379730_500000_CN_168727982_500000 : powerlib/Elements/Distributed Parameters Line  Phases=3  Frequency=50  Resistance=[0.01273 0.3864]  Inductance="[0.9337e-3  4.1264e-3]"  Capacitance=[12.74e-9 7.751e-9]  Length=49.2834  x1=[8.73114913702011e-11 380000 380000;314.159265358979 314.159265358979 314.159265358979;-0.177670123217348 0.415246442777429 -1.15554988401747]  x2=[1.26090477118469e-09 381852.398472139 381852.398472139;314.159265358979 314.159265358979 314.159265358979;-1.41941675517191 0.415007521738739 -1.15578880505616]  x3=[1.07663708898761e-11 1405.24743813465 1405.24743813466;314.159265358979 314.159265358979 314.159265358979;-2.70558821102223 0.316110507002444 -1.25468581979246]  x4=[8.62234243168895e-12 1405.96374414071 1405.9637441407;314.159265358979 314.159265358979 314.159265358979;0.245769282942371 0.405640215255436 -1.16515611153945]  x5=0.000565541566995742  V1=ones(3,3)  V2=ones(3,3)  I1=ones(3,3)  I2=ones(3,3)  nHarmo=1  Measurements=None
  新京葉線_CN_133135172_500000_CN_168727982_500000 : powerlib/Elements/Distributed Parameters Line  Phases=3  Frequency=50  Resistance=[0.01273 0.3864]  Inductance="[0.9337e-3  4.1264e-3]"  Capacitance=[12.74e-9 7.751e-9]  Length=56.7083  x1=[8.73114913702011e-11 380000 380000;314.159265358979 314.159265358979 314.159265358979;-0.177670123217348 0.415246442777429 -1.15554988401747]  x2=[1.26090477118469e-09 381852.398472139 381852.398472139;314.159265358979 314.159265358979 314.159265358979;-1.41941675517191 0.415007521738739 -1.15578880505616]  x3=[1.07663708898761e-11 1405.24743813465 1405.24743813466;314.159265358979 314.159265358979 314.159265358979;-2.70558821102223 0.316110507002444 -1.25468581979246]  x4=[8.62234243168895e-12 1405.96374414071 1405.9637441407;314.159265358979 314.159265358979 314.159265358979;0.245769282942371 0.405640215255436 -1.16515611153945]  x5=0.000565541566995742  V1=ones(3,3)  V2=ones(3,3)  I1=ones(3,3)  I2=ones(3,3)  nHarmo=1  Measurements=None
  新古河線_(Shin_Koga_Sen)_CN_133135172_500000_CN_133641619_500000 : powerlib/Elements/Distributed Parameters Line  Phases=3  Frequency=50  Resistance=[0.01273 0.3864]  Inductance="[0.9337e-3  4.1264e-3]"  Capacitance=[12.74e-9 7.751e-9]  Length=70.1875  x1=[8.73114913702011e-11 380000 380000;314.159265358979 314.159265358979 314.159265358979;-0.177670123217348 0.415246442777429 -1.15554988401747]  x2=[1.26090477118469e-09 381852.398472139 381852.398472139;314.159265358979 314.159265358979 314.159265358979;-1.41941675517191 0.415007521738739 -1.15578880505616]  x3=[1.07663708898761e-11 1405.24743813465 1405.24743813466;314.159265358979 314.159265358979 314.159265358979;-2.70558821102223 0.316110507002444 -1.25468581979246]  x4=[8.62234243168895e-12 1405.96374414071 1405.9637441407;314.159265358979 314.159265358979 314.159265358979;0.245769282942371 0.405640215255436 -1.16515611153945]  x5=0.000565541566995742  V1=ones(3,3)  V2=ones(3,3)  I1=ones(3,3)  I2=ones(3,3)  nHarmo=1  Measurements=None
  新坂戸線_CN_128581912_500000_CN_133641619_500000 : powerlib/Elements/Distributed Parameters Line  Phases=3  Frequency=50  Resistance=[0.01273 0.3864]  Inductance="[0.9337e-3  4.1264e-3]"  Capacitance=[12.74e-9 7.751e-9]  Length=8.954  x1=[8.73114913702011e-11 380000 380000;314.159265358979 314.159265358979 314.159265358979;-0.177670123217348 0.415246442777429 -1.15554988401747]  x2=[1.26090477118469e-09 381852.398472139 381852.398472139;314.159265358979 314.159265358979 314.159265358979;-1.41941675517191 0.415007521738739 -1.15578880505616]  x3=[1.07663708898761e-11 1405.24743813465 1405.24743813466;314.159265358979 314.159265358979 314.159265358979;-2.70558821102223 0.316110507002444 -1.25468581979246]  x4=[8.62234243168895e-12 1405.96374414071 1405.9637441407;314.159265358979 314.159265358979 314.159265358979;0.245769282942371 0.405640215255436 -1.16515611153945]  x5=0.000565541566995742  V1=ones(3,3)  V2=ones(3,3)  I1=ones(3,3)  I2=ones(3,3)  nHarmo=1  Measurements=None
  新多摩線_(Shin_Tama_Sen)_CN_149843487_500000_CN_145079972_500000 : powerlib/Elements/Distributed Parameters Line  Phases=3  Frequency=50  Resistance=[0.01273 0.3864]  Inductance="[0.9337e-3  4.1264e-3]"  Capacitance=[12.74e-9 7.751e-9]  Length=49.1338  x1=[8.73114913702011e-11 380000 380000;314.159265358979 314.159265358979 314.159265358979;-0.177670123217348 0.415246442777429 -1.15554988401747]  x2=[1.26090477118469e-09 381852.398472139 381852.398472139;314.159265358979 314.159265358979 314.159265358979;-1.41941675517191 0.415007521738739 -1.15578880505616]  x3=[1.07663708898761e-11 1405.24743813465 1405.24743813466;314.159265358979 314.159265358979 314.159265358979;-2.70558821102223 0.316110507002444 -1.25468581979246]  x4=[8.62234243168895e-12 1405.96374414071 1405.9637441407;314.159265358979 314.159265358979 314.159265358979;0.245769282942371 0.405640215255436 -1.16515611153945]  x5=0.000565541566995742  V1=ones(3,3)  V2=ones(3,3)  I1=ones(3,3)  I2=ones(3,3)  nHarmo=1  Measurements=None
  新所沢線_(Shin_Tokorozawa_Sen)_CN_133641619_500000_CN_145079972_500000 : powerlib/Elements/Distributed Parameters Line  Phases=3  Frequency=50  Resistance=[0.01273 0.3864]  Inductance="[0.9337e-3  4.1264e-3]"  Capacitance=[12.74e-9 7.751e-9]  Length=42.9234  x1=[8.73114913702011e-11 380000 380000;314.159265358979 314.159265358979 314.159265358979;-0.177670123217348 0.415246442777429 -1.15554988401747]  x2=[1.26090477118469e-09 381852.398472139 381852.398472139;314.159265358979 314.159265358979 314.159265358979;-1.41941675517191 0.415007521738739 -1.15578880505616]  x3=[1.07663708898761e-11 1405.24743813465 1405.24743813466;314.159265358979 314.159265358979 314.159265358979;-2.70558821102223 0.316110507002444 -1.25468581979246]  x4=[8.62234243168895e-12 1405.96374414071 1405.9637441407;314.159265358979 314.159265358979 314.159265358979;0.245769282942371 0.405640215255436 -1.16515611153945]  x5=0.000565541566995742  V1=ones(3,3)  V2=ones(3,3)  I1=ones(3,3)  I2=ones(3,3)  nHarmo=1  Measurements=None
  新榛名線_CN_169963227_500000_CN_195615141_500000 : powerlib/Elements/Distributed Parameters Line  Phases=3  Frequency=50  Resistance=[0.01273 0.3864]  Inductance="[0.9337e-3  4.1264e-3]"  Capacitance=[12.74e-9 7.751e-9]  Length=84.221  x1=[8.73114913702011e-11 380000 380000;314.159265358979 314.159265358979 314.159265358979;-0.177670123217348 0.415246442777429 -1.15554988401747]  x2=[1.26090477118469e-09 381852.398472139 381852.398472139;314.159265358979 314.159265358979 314.159265358979;-1.41941675517191 0.415007521738739 -1.15578880505616]  x3=[1.07663708898761e-11 1405.24743813465 1405.24743813466;314.159265358979 314.159265358979 314.159265358979;-2.70558821102223 0.316110507002444 -1.25468581979246]  x4=[8.62234243168895e-12 1405.96374414071 1405.9637441407;314.159265358979 314.159265358979 314.159265358979;0.245769282942371 0.405640215255436 -1.16515611153945]  x5=0.000565541566995742  V1=ones(3,3)  V2=ones(3,3)  I1=ones(3,3)  I2=ones(3,3)  nHarmo=1  Measurements=None
  新筑波線_(Shin_Tsukuba_Sen)_CN_133135172_500000_CN_132913106_500000 : powerlib/Elements/Distributed Parameters Line  Phases=3  Frequency=50  Resistance=[0.01273 0.3864]  Inductance="[0.9337e-3  4.1264e-3]"  Capacitance=[12.74e-9 7.751e-9]  Length=11.623  x1=[8.73114913702011e-11 380000 380000;314.159265358979 314.159265358979 314.159265358979;-0.177670123217348 0.415246442777429 -1.15554988401747]  x2=[1.26090477118469e-09 381852.398472139 381852.398472139;314.159265358979 314.159265358979 314.159265358979;-1.41941675517191 0.415007521738739 -1.15578880505616]  x3=[1.07663708898761e-11 1405.24743813465 1405.24743813466;314.159265358979 314.159265358979 314.159265358979;-2.70558821102223 0.316110507002444 -1.25468581979246]  x4=[8.62234243168895e-12 1405.96374414071 1405.9637441407;314.159265358979 314.159265358979 314.159265358979;0.245769282942371 0.405640215255436 -1.16515611153945]  x5=0.000565541566995742  V1=ones(3,3)  V2=ones(3,3)  I1=ones(3,3)  I2=ones(3,3)  nHarmo=1  Measurements=None
  東京中線_CN_128581912_275000_CN_133137636_275000 : powerlib/Elements/Distributed Parameters Line  Phases=3  Frequency=50  Resistance=[0.01273 0.3864]  Inductance="[0.9337e-3  4.1264e-3]"  Capacitance=[12.74e-9 7.751e-9]  Length=31.3603  x1=[8.73114913702011e-11 380000 380000;314.159265358979 314.159265358979 314.159265358979;-0.177670123217348 0.415246442777429 -1.15554988401747]  x2=[1.26090477118469e-09 381852.398472139 381852.398472139;314.159265358979 314.159265358979 314.159265358979;-1.41941675517191 0.415007521738739 -1.15578880505616]  x3=[1.07663708898761e-11 1405.24743813465 1405.24743813466;314.159265358979 314.159265358979 314.159265358979;-2.70558821102223 0.316110507002444 -1.25468581979246]  x4=[8.62234243168895e-12 1405.96374414071 1405.9637441407;314.159265358979 314.159265358979 314.159265358979;0.245769282942371 0.405640215255436 -1.16515611153945]  x5=0.000565541566995742  V1=ones(3,3)  V2=ones(3,3)  I1=ones(3,3)  I2=ones(3,3)  nHarmo=1  Measurements=None
  東京南線3;4号線_CN_128364781_275000_CN379474501 : powerlib/Elements/Distributed Parameters Line  Phases=3  Frequency=50  Resistance=[0.01273 0.3864]  Inductance="[0.9337e-3  4.1264e-3]"  Capacitance=[12.74e-9 7.751e-9]  Length=43.4198  x1=[8.73114913702011e-11 380000 380000;314.159265358979 314.159265358979 314.159265358979;-0.177670123217348 0.415246442777429 -1.15554988401747]  x2=[1.26090477118469e-09 381852.398472139 381852.398472139;314.159265358979 314.159265358979 314.159265358979;-1.41941675517191 0.415007521738739 -1.15578880505616]  x3=[1.07663708898761e-11 1405.24743813465 1405.24743813466;314.159265358979 314.159265358979 314.159265358979;-2.70558821102223 0.316110507002444 -1.25468581979246]  x4=[8.62234243168895e-12 1405.96374414071 1405.9637441407;314.159265358979 314.159265358979 314.159265358979;0.245769282942371 0.405640215255436 -1.16515611153945]  x5=0.000565541566995742  V1=ones(3,3)  V2=ones(3,3)  I1=ones(3,3)  I2=ones(3,3)  nHarmo=1  Measurements=None
  東京西線_CN_145080115_275000_CN_47110637_275000 : powerlib/Elements/Distributed Parameters Line  Phases=3  Frequency=50  Resistance=[0.01273 0.3864]  Inductance="[0.9337e-3  4.1264e-3]"  Capacitance=[12.74e-9 7.751e-9]  Length=16.2597  x1=[8.73114913702011e-11 380000 380000;314.159265358979 314.159265358979 314.159265358979;-0.177670123217348 0.415246442777429 -1.15554988401747]  x2=[1.26090477118469e-09 381852.398472139 381852.398472139;314.159265358979 314.159265358979 314.159265358979;-1.41941675517191 0.415007521738739 -1.15578880505616]  x3=[1.07663708898761e-11 1405.24743813465 1405.24743813466;314.159265358979 314.159265358979 314.159265358979;-2.70558821102223 0.316110507002444 -1.25468581979246]  x4=[8.62234243168895e-12 1405.96374414071 1405.9637441407;314.159265358979 314.159265358979 314.159265358979;0.245769282942371 0.405640215255436 -1.16515611153945]  x5=0.000565541566995742  V1=ones(3,3)  V2=ones(3,3)  I1=ones(3,3)  I2=ones(3,3)  nHarmo=1  Measurements=None
  東群馬幹線_CN_250540807_500000_CN_66098469_500000 : powerlib/Elements/Distributed Parameters Line  Phases=3  Frequency=50  Resistance=[0.01273 0.3864]  Inductance="[0.9337e-3  4.1264e-3]"  Capacitance=[12.74e-9 7.751e-9]  Length=55.3432  x1=[8.73114913702011e-11 380000 380000;314.159265358979 314.159265358979 314.159265358979;-0.177670123217348 0.415246442777429 -1.15554988401747]  x2=[1.26090477118469e-09 381852.398472139 381852.398472139;314.159265358979 314.159265358979 314.159265358979;-1.41941675517191 0.415007521738739 -1.15578880505616]  x3=[1.07663708898761e-11 1405.24743813465 1405.24743813466;314.159265358979 314.159265358979 314.159265358979;-2.70558821102223 0.316110507002444 -1.25468581979246]  x4=[8.62234243168895e-12 1405.96374414071 1405.9637441407;314.159265358979 314.159265358979 314.159265358979;0.245769282942371 0.405640215255436 -1.16515611153945]  x5=0.000565541566995742  V1=ones(3,3)  V2=ones(3,3)  I1=ones(3,3)  I2=ones(3,3)  nHarmo=1  Measurements=None
  泉南東大阪線_(Sennan_Higashiōsaka_sen)_CN_108199478_275000_CN_158522649_275000 : powerlib/Elements/Distributed Parameters Line  Phases=3  Frequency=50  Resistance=[0.01273 0.3864]  Inductance="[0.9337e-3  4.1264e-3]"  Capacitance=[12.74e-9 7.751e-9]  Length=52.783  x1=[8.73114913702011e-11 380000 380000;314.159265358979 314.159265358979 314.159265358979;-0.177670123217348 0.415246442777429 -1.15554988401747]  x2=[1.26090477118469e-09 381852.398472139 381852.398472139;314.159265358979 314.159265358979 314.159265358979;-1.41941675517191 0.415007521738739 -1.15578880505616]  x3=[1.07663708898761e-11 1405.24743813465 1405.24743813466;314.159265358979 314.159265358979 314.159265358979;-2.70558821102223 0.316110507002444 -1.25468581979246]  x4=[8.62234243168895e-12 1405.96374414071 1405.9637441407;314.159265358979 314.159265358979 314.159265358979;0.245769282942371 0.405640215255436 -1.16515611153945]  x5=0.000565541566995742  V1=ones(3,3)  V2=ones(3,3)  I1=ones(3,3)  I2=ones(3,3)  nHarmo=1  Measurements=None
  湖西三河線_CN_170247308_275000_CN_170260165_275000 : powerlib/Elements/Distributed Parameters Line  Phases=3  Frequency=50  Resistance=[0.01273 0.3864]  Inductance="[0.9337e-3  4.1264e-3]"  Capacitance=[12.74e-9 7.751e-9]  Length=21.1768  x1=[8.73114913702011e-11 380000 380000;314.159265358979 314.159265358979 314.159265358979;-0.177670123217348 0.415246442777429 -1.15554988401747]  x2=[1.26090477118469e-09 381852.398472139 381852.398472139;314.159265358979 314.159265358979 314.159265358979;-1.41941675517191 0.415007521738739 -1.15578880505616]  x3=[1.07663708898761e-11 1405.24743813465 1405.24743813466;314.159265358979 314.159265358979 314.159265358979;-2.70558821102223 0.316110507002444 -1.25468581979246]  x4=[8.62234243168895e-12 1405.96374414071 1405.9637441407;314.159265358979 314.159265358979 314.159265358979;0.245769282942371 0.405640215255436 -1.16515611153945]  x5=0.000565541566995742  V1=ones(3,3)  V2=ones(3,3)  I1=ones(3,3)  I2=ones(3,3)  nHarmo=1  Measurements=None
  福島東幹線2_CN_106309481_500000_CN_104391636_500000 : powerlib/Elements/Distributed Parameters Line  Phases=3  Frequency=50  Resistance=[0.01273 0.3864]  Inductance="[0.9337e-3  4.1264e-3]"  Capacitance=[12.74e-9 7.751e-9]  Length=41.6249  x1=[8.73114913702011e-11 380000 380000;314.159265358979 314.159265358979 314.159265358979;-0.177670123217348 0.415246442777429 -1.15554988401747]  x2=[1.26090477118469e-09 381852.398472139 381852.398472139;314.159265358979 314.159265358979 314.159265358979;-1.41941675517191 0.415007521738739 -1.15578880505616]  x3=[1.07663708898761e-11 1405.24743813465 1405.24743813466;314.159265358979 314.159265358979 314.159265358979;-2.70558821102223 0.316110507002444 -1.25468581979246]  x4=[8.62234243168895e-12 1405.96374414071 1405.9637441407;314.159265358979 314.159265358979 314.159265358979;0.245769282942371 0.405640215255436 -1.16515611153945]  x5=0.000565541566995742  V1=ones(3,3)  V2=ones(3,3)  I1=ones(3,3)  I2=ones(3,3)  nHarmo=1  Measurements=None
  秦浜線_CN_162844704_275000_CN_128364781_275000 : powerlib/Elements/Distributed Parameters Line  Phases=3  Frequency=50  Resistance=[0.01273 0.3864]  Inductance="[0.9337e-3  4.1264e-3]"  Capacitance=[12.74e-9 7.751e-9]  Length=11.116  x1=[8.73114913702011e-11 380000 380000;314.159265358979 314.159265358979 314.159265358979;-0.177670123217348 0.415246442777429 -1.15554988401747]  x2=[1.26090477118469e-09 381852.398472139 381852.398472139;314.159265358979 314.159265358979 314.159265358979;-1.41941675517191 0.415007521738739 -1.15578880505616]  x3=[1.07663708898761e-11 1405.24743813465 1405.24743813466;314.159265358979 314.159265358979 314.159265358979;-2.70558821102223 0.316110507002444 -1.25468581979246]  x4=[8.62234243168895e-12 1405.96374414071 1405.9637441407;314.159265358979 314.159265358979 314.159265358979;0.245769282942371 0.405640215255436 -1.16515611153945]  x5=0.000565541566995742  V1=ones(3,3)  V2=ones(3,3)  I1=ones(3,3)  I2=ones(3,3)  nHarmo=1  Measurements=None
  西越谷線_(Nishi_Koshigaya_Sen)_CN_153521822_275000_CN_133137636_275000 : powerlib/Elements/Distributed Parameters Line  Phases=3  Frequency=50  Resistance=[0.01273 0.3864]  Inductance="[0.9337e-3  4.1264e-3]"  Capacitance=[12.74e-9 7.751e-9]  Length=21.7767  x1=[8.73114913702011e-11 380000 380000;314.159265358979 314.159265358979 314.159265358979;-0.177670123217348 0.415246442777429 -1.15554988401747]  x2=[1.26090477118469e-09 381852.398472139 381852.398472139;314.159265358979 314.159265358979 314.159265358979;-1.41941675517191 0.415007521738739 -1.15578880505616]  x3=[1.07663708898761e-11 1405.24743813465 1405.24743813466;314.159265358979 314.159265358979 314.159265358979;-2.70558821102223 0.316110507002444 -1.25468581979246]  x4=[8.62234243168895e-12 1405.96374414071 1405.9637441407;314.159265358979 314.159265358979 314.159265358979;0.245769282942371 0.405640215255436 -1.16515611153945]  x5=0.000565541566995742  V1=ones(3,3)  V2=ones(3,3)  I1=ones(3,3)  I2=ones(3,3)  nHarmo=1  Measurements=None
  豊根幹線_CN_170850727_500000_CN_142662111_500000 : powerlib/Elements/Distributed Parameters Line  Phases=3  Frequency=50  Resistance=[0.01273 0.3864]  Inductance="[0.9337e-3  4.1264e-3]"  Capacitance=[12.74e-9 7.751e-9]  Length=53.0192  x1=[8.73114913702011e-11 380000 380000;314.159265358979 314.159265358979 314.159265358979;-0.177670123217348 0.415246442777429 -1.15554988401747]  x2=[1.26090477118469e-09 381852.398472139 381852.398472139;314.159265358979 314.159265358979 314.159265358979;-1.41941675517191 0.415007521738739 -1.15578880505616]  x3=[1.07663708898761e-11 1405.24743813465 1405.24743813466;314.159265358979 314.159265358979 314.159265358979;-2.70558821102223 0.316110507002444 -1.25468581979246]  x4=[8.62234243168895e-12 1405.96374414071 1405.9637441407;314.159265358979 314.159265358979 314.159265358979;0.245769282942371 0.405640215255436 -1.16515611153945]  x5=0.000565541566995742  V1=ones(3,3)  V2=ones(3,3)  I1=ones(3,3)  I2=ones(3,3)  nHarmo=1  Measurements=None
  金剛線_(Kongō_sen)_CN_109834508_275000_CN_291678103_275000 : powerlib/Elements/Distributed Parameters Line  Phases=3  Frequency=50  Resistance=[0.01273 0.3864]  Inductance="[0.9337e-3  4.1264e-3]"  Capacitance=[12.74e-9 7.751e-9]  Length=50.4928  x1=[8.73114913702011e-11 380000 380000;314.159265358979 314.159265358979 314.159265358979;-0.177670123217348 0.415246442777429 -1.15554988401747]  x2=[1.26090477118469e-09 381852.398472139 381852.398472139;314.159265358979 314.159265358979 314.159265358979;-1.41941675517191 0.415007521738739 -1.15578880505616]  x3=[1.07663708898761e-11 1405.24743813465 1405.24743813466;314.159265358979 314.159265358979 314.159265358979;-2.70558821102223 0.316110507002444 -1.25468581979246]  x4=[8.62234243168895e-12 1405.96374414071 1405.9637441407;314.159265358979 314.159265358979 314.159265358979;0.245769282942371 0.405640215255436 -1.16515611153945]  x5=0.000565541566995742  V1=ones(3,3)  V2=ones(3,3)  I1=ones(3,3)  I2=ones(3,3)  nHarmo=1  Measurements=None
  関門連系線_CN_204258596_500000_CN_187988970_500000 : powerlib/Elements/Distributed Parameters Line  Phases=3  Frequency=50  Resistance=[0.01273 0.3864]  Inductance="[0.9337e-3  4.1264e-3]"  Capacitance=[12.74e-9 7.751e-9]  Length=77.4957  x1=[8.73114913702011e-11 380000 380000;314.159265358979 314.159265358979 314.159265358979;-0.177670123217348 0.415246442777429 -1.15554988401747]  x2=[1.26090477118469e-09 381852.398472139 381852.398472139;314.159265358979 314.159265358979 314.159265358979;-1.41941675517191 0.415007521738739 -1.15578880505616]  x3=[1.07663708898761e-11 1405.24743813465 1405.24743813466;314.159265358979 314.159265358979 314.159265358979;-2.70558821102223 0.316110507002444 -1.25468581979246]  x4=[8.62234243168895e-12 1405.96374414071 1405.9637441407;314.159265358979 314.159265358979 314.159265358979;0.245769282942371 0.405640215255436 -1.16515611153945]  x5=0.000565541566995742  V1=ones(3,3)  V2=ones(3,3)  I1=ones(3,3)  I2=ones(3,3)  nHarmo=1  Measurements=None
  阿南紀北直流幹線_CN_109850439_500000_CN_217885658_500000 : powerlib/Elements/Distributed Parameters Line  Phases=3  Frequency=50  Resistance=[0.01273 0.3864]  Inductance="[0.9337e-3  4.1264e-3]"  Capacitance=[12.74e-9 7.751e-9]  Length=61.602  x1=[8.73114913702011e-11 380000 380000;314.159265358979 314.159265358979 314.159265358979;-0.177670123217348 0.415246442777429 -1.15554988401747]  x2=[1.26090477118469e-09 381852.398472139 381852.398472139;314.159265358979 314.159265358979 314.159265358979;-1.41941675517191 0.415007521738739 -1.15578880505616]  x3=[1.07663708898761e-11 1405.24743813465 1405.24743813466;314.159265358979 314.159265358979 314.159265358979;-2.70558821102223 0.316110507002444 -1.25468581979246]  x4=[8.62234243168895e-12 1405.96374414071 1405.9637441407;314.159265358979 314.159265358979 314.159265358979;0.245769282942371 0.405640215255436 -1.16515611153945]  x5=0.000565541566995742  V1=ones(3,3)  V2=ones(3,3)  I1=ones(3,3)  I2=ones(3,3)  nHarmo=1  Measurements=None
  駿遠幹線_CN_116559939_500000_CN_210090094_500000 : powerlib/Elements/Distributed Parameters Line  Phases=3  Frequency=50  Resistance=[0.01273 0.3864]  Inductance="[0.9337e-3  4.1264e-3]"  Capacitance=[12.74e-9 7.751e-9]  Length=56.5258  x1=[8.73114913702011e-11 380000 380000;314.159265358979 314.159265358979 314.159265358979;-0.177670123217348 0.415246442777429 -1.15554988401747]  x2=[1.26090477118469e-09 381852.398472139 381852.398472139;314.159265358979 314.159265358979 314.159265358979;-1.41941675517191 0.415007521738739 -1.15578880505616]  x3=[1.07663708898761e-11 1405.24743813465 1405.24743813466;314.159265358979 314.159265358979 314.159265358979;-2.70558821102223 0.316110507002444 -1.25468581979246]  x4=[8.62234243168895e-12 1405.96374414071 1405.9637441407;314.159265358979 314.159265358979 314.159265358979;0.245769282942371 0.405640215255436 -1.16515611153945]  x5=0.000565541566995742  V1=ones(3,3)  V2=ones(3,3)  I1=ones(3,3)  I2=ones(3,3)  nHarmo=1  Measurements=None
  connections:
  _CN_201293312_500000_CN_216778426_500000/LConn1 -- T_201293312_500000;220000_/LConn1 -- _CN_201293312_500000_CN_187988970_500000/LConn1
  _CN_201293312_500000_CN_216778426_500000/LConn2 -- T_201293312_500000;220000_/LConn2 -- _CN_201293312_500000_CN_187988970_500000/LConn2
  _CN_201293312_500000_CN_216778426_500000/LConn3 -- T_201293312_500000;220000_/LConn3 -- _CN_201293312_500000_CN_187988970_500000/LConn3
  T_216778426_500000;220000_/LConn1 -- _CN_201293312_500000_CN_216778426_500000/RConn1
  T_216778426_500000;220000_/LConn2 -- _CN_201293312_500000_CN_216778426_500000/RConn2
  T_216778426_500000;220000_/LConn3 -- _CN_201293312_500000_CN_216778426_500000/RConn3
  _CN_201293312_500000_CN_187988970_500000/RConn1 -- T_187988970_500000;220000_/LConn1 -- 関門連系線_CN_204258596_500000_CN_187988970_500000/LConn1
  _CN_201293312_500000_CN_187988970_500000/RConn2 -- T_187988970_500000;220000_/LConn2 -- 関門連系線_CN_204258596_500000_CN_187988970_500000/LConn2
  _CN_201293312_500000_CN_187988970_500000/RConn3 -- T_187988970_500000;220000_/LConn3 -- 関門連系線_CN_204258596_500000_CN_187988970_500000/LConn3
  T_104173570_500000_/LConn1 -- _CN_104173570_500000_CN_106309481_500000/LConn1
  T_104173570_500000_/LConn2 -- _CN_104173570_500000_CN_106309481_500000/LConn2
  T_104173570_500000_/LConn3 -- _CN_104173570_500000_CN_106309481_500000/LConn3
  _CN_104173570_500000_CN_106309481_500000/RConn1 -- T_106309481_500000_新福島変電所/LConn1 -- 福島東幹線2_CN_106309481_500000_CN_104391636_500000/LConn1 -- _CN_106309481_500000_CN103783431/LConn1
  _CN_104173570_500000_CN_106309481_500000/RConn2 -- T_106309481_500000_新福島変電所/LConn2 -- 福島東幹線2_CN_106309481_500000_CN_104391636_500000/LConn2 -- _CN_106309481_500000_CN103783431/LConn2
  _CN_104173570_500000_CN_106309481_500000/RConn3 -- T_106309481_500000_新福島変電所/LConn3 -- 福島東幹線2_CN_106309481_500000_CN_104391636_500000/LConn3 -- _CN_106309481_500000_CN103783431/LConn3
  T_116828675_275000_北相模変電所_(Kita_Sagami_Hendensho)/LConn1 -- 佐久間東幹線_CN_116828675_275000_CN134376414/LConn1
  T_116828675_275000_北相模変電所_(Kita_Sagami_Hendensho)/LConn2 -- 佐久間東幹線_CN_116828675_275000_CN134376414/LConn2
  T_116828675_275000_北相模変電所_(Kita_Sagami_Hendensho)/LConn3 -- 佐久間東幹線_CN_116828675_275000_CN134376414/LConn3
  G_134376414_佐久間発電所/RConn1 -- 佐久間東幹線_CN_116828675_275000_CN134376414/RConn1
  G_134376414_佐久間発電所/RConn2 -- 佐久間東幹線_CN_116828675_275000_CN134376414/RConn2
  G_134376414_佐久間発電所/RConn3 -- 佐久間東幹線_CN_116828675_275000_CN134376414/RConn3
  T_169121284_275000_/LConn1 -- _CN_169121284_275000_CN_169121278_275000/LConn1
  T_169121284_275000_/LConn2 -- _CN_169121284_275000_CN_169121278_275000/LConn2
  T_169121284_275000_/LConn3 -- _CN_169121284_275000_CN_169121278_275000/LConn3
  _CN_169121284_275000_CN_169121278_275000/RConn1 -- T_169121278_275000_電源名古屋/LConn1 -- _CN_170366038_275000_CN_169121278_275000/LConn1
  _CN_169121284_275000_CN_169121278_275000/RConn2 -- T_169121278_275000_電源名古屋/LConn2 -- _CN_170366038_275000_CN_169121278_275000/LConn2
  _CN_169121284_275000_CN_169121278_275000/RConn3 -- T_169121278_275000_電源名古屋/LConn3 -- _CN_170366038_275000_CN_169121278_275000/LConn3
  _CN_193544791_500000_CN_170974371_500000/LConn1 -- T_193544791_500000_新西広島変電所_(Shin_Nishi_Hiroshima_Hendensho)/LConn1 -- _CN_193544791_500000_CN_242253500_500000/LConn1 -- _CN_193544791_500000_CN_317416612_500000/LConn1
  _CN_193544791_500000_CN_170974371_500000/LConn2 -- T_193544791_500000_新西広島変電所_(Shin_Nishi_Hiroshima_Hendensho)/LConn2 -- _CN_193544791_500000_CN_242253500_500000/LConn2 -- _CN_193544791_500000_CN_317416612_500000/LConn2
  _CN_193544791_500000_CN_170974371_500000/LConn3 -- T_193544791_500000_新西広島変電所_(Shin_Nishi_Hiroshima_Hendensho)/LConn3 -- _CN_193544791_500000_CN_242253500_500000/LConn3 -- _CN_193544791_500000_CN_317416612_500000/LConn3
  _CN_193544791_500000_CN_170974371_500000/RConn1 -- T_170974371_500000_新広島変電所_(Shin_Hiroshima_Hendensho)/LConn1 -- _CN_170974371_500000_CN_241828221_500000/LConn1
  _CN_193544791_500000_CN_170974371_500000/RConn2 -- T_170974371_500000_新広島変電所_(Shin_Hiroshima_Hendensho)/LConn2 -- _CN_170974371_500000_CN_241828221_500000/LConn2
  _CN_193544791_500000_CN_170974371_500000/RConn3 -- T_170974371_500000_新広島変電所_(Shin_Hiroshima_Hendensho)/LConn3 -- _CN_170974371_500000_CN_241828221_500000/LConn3
  _CN_193544791_500000_CN_242253500_500000/RConn1 -- T_242253500_500000_東山口変電所_(Higashi_Yamaguchi_Hendensho)/LConn1 -- _CN_242253500_500000_CN_204258596_500000/LConn1
  _CN_193544791_500000_CN_242253500_500000/RConn2 -- T_242253500_500000_東山口変電所_(Higashi_Yamaguchi_Hendensho)/LConn2 -- _CN_242253500_500000_CN_204258596_500000/LConn2
  _CN_193544791_500000_CN_242253500_500000/RConn3 -- T_242253500_500000_東山口変電所_(Higashi_Yamaguchi_Hendensho)/LConn3 -- _CN_242253500_500000_CN_204258596_500000/LConn3
  _CN_193544791_500000_CN_317416612_500000/RConn1 -- T_317416612_500000_西島根変電所/LConn1 -- _CN_317416612_500000_CN_204258596_500000/LConn1 -- _CN_242103481_500000_CN_317416612_500000/LConn1
  _CN_193544791_500000_CN_317416612_500000/RConn2 -- T_317416612_500000_西島根変電所/LConn2 -- _CN_317416612_500000_CN_204258596_500000/LConn2 -- _CN_242103481_500000_CN_317416612_500000/LConn2
  _CN_193544791_500000_CN_317416612_500000/RConn3 -- T_317416612_500000_西島根変電所/LConn3 -- _CN_317416612_500000_CN_204258596_500000/LConn3 -- _CN_242103481_500000_CN_317416612_500000/LConn3
  _CN_161727149_500000_CN_169031921_500000/LConn1 -- T_161727149_500000_新生駒変電所_(Shin_Ikoma_Hendensho)/LConn1 -- _CN_161727149_500000_CN_161870227_500000/LConn1 -- _CN_161727149_500000_CN_169359724_500000/LConn1
  _CN_161727149_500000_CN_169031921_500000/LConn2 -- T_161727149_500000_新生駒変電所_(Shin_Ikoma_Hendensho)/LConn2 -- _CN_161727149_500000_CN_161870227_500000/LConn2 -- _CN_161727149_500000_CN_169359724_500000/LConn2
  _CN_161727149_500000_CN_169031921_500000/LConn3 -- T_161727149_500000_新生駒変電所_(Shin_Ikoma_Hendensho)/LConn3 -- _CN_161727149_500000_CN_161870227_500000/LConn3 -- _CN_161727149_500000_CN_169359724_500000/LConn3
  _CN_161727149_500000_CN_169031921_500000/RConn1 -- T_169031921_500000_西京都変電所_(Nishi_Kyōto_Hendensho)/LConn1 -- _CN_320438391_500000_CN_169031921_500000/LConn1
  _CN_161727149_500000_CN_169031921_500000/RConn2 -- T_169031921_500000_西京都変電所_(Nishi_Kyōto_Hendensho)/LConn2 -- _CN_320438391_500000_CN_169031921_500000/LConn2
  _CN_161727149_500000_CN_169031921_500000/RConn3 -- T_169031921_500000_西京都変電所_(Nishi_Kyōto_Hendensho)/LConn3 -- _CN_320438391_500000_CN_169031921_500000/LConn3
  T_169359724_500000_信貴変電所_(Shingi_Hendensho)/LConn1 -- _CN_161727149_500000_CN_169359724_500000/RConn1
  T_169359724_500000_信貴変電所_(Shingi_Hendensho)/LConn2 -- _CN_161727149_500000_CN_169359724_500000/RConn2
  T_169359724_500000_信貴変電所_(Shingi_Hendensho)/LConn3 -- _CN_161727149_500000_CN_169359724_500000/RConn3
  _CN_161727149_500000_CN_161870227_500000/RConn1 -- T_161870227_500000_南京都変電所_(Minami_Kyōto_Hendensho)/LConn1 -- _CN_170589736_500000_CN_161870227_500000/LConn1
  _CN_161727149_500000_CN_161870227_500000/RConn2 -- T_161870227_500000_南京都変電所_(Minami_Kyōto_Hendensho)/LConn2 -- _CN_170589736_500000_CN_161870227_500000/LConn2
  _CN_161727149_500000_CN_161870227_500000/RConn3 -- T_161870227_500000_南京都変電所_(Minami_Kyōto_Hendensho)/LConn3 -- _CN_170589736_500000_CN_161870227_500000/LConn3
  _CN_149843487_500000_CN_150065045_500000/LConn1 -- T_149843487_500000_新秦野変電所_(Shin_Hatano_Hendensho)/LConn1 -- 新多摩線_(Shin_Tama_Sen)_CN_149843487_500000_CN_145079972_500000/LConn1
  _CN_149843487_500000_CN_150065045_500000/LConn2 -- T_149843487_500000_新秦野変電所_(Shin_Hatano_Hendensho)/LConn2 -- 新多摩線_(Shin_Tama_Sen)_CN_149843487_500000_CN_145079972_500000/LConn2
  _CN_149843487_500000_CN_150065045_500000/LConn3 -- T_149843487_500000_新秦野変電所_(Shin_Hatano_Hendensho)/LConn3 -- 新多摩線_(Shin_Tama_Sen)_CN_149843487_500000_CN_145079972_500000/LConn3
  _CN_149843487_500000_CN_150065045_500000/RConn1 -- T_150065045_500000_新富士変電所/LConn1 -- _CN_150035494_500000_CN_150065045_500000/LConn1
  _CN_149843487_500000_CN_150065045_500000/RConn2 -- T_150065045_500000_新富士変電所/LConn2 -- _CN_150035494_500000_CN_150065045_500000/LConn2
  _CN_149843487_500000_CN_150065045_500000/RConn3 -- T_150065045_500000_新富士変電所/LConn3 -- _CN_150035494_500000_CN_150065045_500000/LConn3
  新多摩線_(Shin_Tama_Sen)_CN_149843487_500000_CN_145079972_500000/RConn1 -- T_145079972_500000_新多摩変電所_(Shin_Tama_Substation)/LConn1 -- 新所沢線_(Shin_Tokorozawa_Sen)_CN_133641619_500000_CN_145079972_500000/LConn1 -- _CN_195615141_500000_CN_145079972_500000/LConn1
  新多摩線_(Shin_Tama_Sen)_CN_149843487_500000_CN_145079972_500000/RConn2 -- T_145079972_500000_新多摩変電所_(Shin_Tama_Substation)/LConn2 -- 新所沢線_(Shin_Tokorozawa_Sen)_CN_133641619_500000_CN_145079972_500000/LConn2 -- _CN_195615141_500000_CN_145079972_500000/LConn2
  新多摩線_(Shin_Tama_Sen)_CN_149843487_500000_CN_145079972_500000/RConn3 -- T_145079972_500000_新多摩変電所_(Shin_Tama_Substation)/LConn3 -- 新所沢線_(Shin_Tokorozawa_Sen)_CN_133641619_500000_CN_145079972_500000/LConn3 -- _CN_195615141_500000_CN_145079972_500000/LConn3
  T_162844704_275000_中相模変電所/LConn1 -- 秦浜線_CN_162844704_275000_CN_128364781_275000/LConn1
  T_162844704_275000_中相模変電所/LConn2 -- 秦浜線_CN_162844704_275000_CN_128364781_275000/LConn2
  T_162844704_275000_中相模変電所/LConn3 -- 秦浜線_CN_162844704_275000_CN_128364781_275000/LConn3
  秦浜線_CN_162844704_275000_CN_128364781_275000/RConn1 -- T_128364781_275000_東京電力_京浜変電所/LConn1 -- 東京南線3;4号線_CN_128364781_275000_CN379474501/LConn1 -- 京浜線1;2号線_CN_128364781_275000_CN_47110637_275000/LConn1
  秦浜線_CN_162844704_275000_CN_128364781_275000/RConn2 -- T_128364781_275000_東京電力_京浜変電所/LConn2 -- 東京南線3;4号線_CN_128364781_275000_CN379474501/LConn2 -- 京浜線1;2号線_CN_128364781_275000_CN_47110637_275000/LConn2
  秦浜線_CN_162844704_275000_CN_128364781_275000/RConn3 -- T_128364781_275000_東京電力_京浜変電所/LConn3 -- 東京南線3;4号線_CN_128364781_275000_CN379474501/LConn3 -- 京浜線1;2号線_CN_128364781_275000_CN_47110637_275000/LConn3
  _CN_150035494_500000_CN216480979/LConn1 -- T_150035494_500000_/LConn1 -- _CN_150035494_500000_CN_66098469_500000/LConn1 -- _CN_150035494_500000_CN_150065045_500000/RConn1
  _CN_150035494_500000_CN216480979/LConn2 -- T_150035494_500000_/LConn2 -- _CN_150035494_500000_CN_66098469_500000/LConn2 -- _CN_150035494_500000_CN_150065045_500000/RConn2
  _CN_150035494_500000_CN216480979/LConn3 -- T_150035494_500000_/LConn3 -- _CN_150035494_500000_CN_66098469_500000/LConn3 -- _CN_150035494_500000_CN_150065045_500000/RConn3
  _CN_150035494_500000_CN216480979/RConn1 -- G_216480979_柏崎刈羽原子力発電所/RConn1 -- _CN_66098469_500000_CN216480979/LConn1
  _CN_150035494_500000_CN216480979/RConn2 -- G_216480979_柏崎刈羽原子力発電所/RConn2 -- _CN_66098469_500000_CN216480979/LConn2
  _CN_150035494_500000_CN216480979/RConn3 -- G_216480979_柏崎刈羽原子力発電所/RConn3 -- _CN_66098469_500000_CN216480979/LConn3
  _CN_150035494_500000_CN_66098469_500000/RConn1 -- T_66098469_500000_西群馬開閉所/LConn1 -- 東群馬幹線_CN_250540807_500000_CN_66098469_500000/LConn1 -- _CN_66098469_500000_CN216480979/RConn1
  _CN_150035494_500000_CN_66098469_500000/RConn2 -- T_66098469_500000_西群馬開閉所/LConn2 -- 東群馬幹線_CN_250540807_500000_CN_66098469_500000/LConn2 -- _CN_66098469_500000_CN216480979/RConn2
  _CN_150035494_500000_CN_66098469_500000/RConn3 -- T_66098469_500000_西群馬開閉所/LConn3 -- 東群馬幹線_CN_250540807_500000_CN_66098469_500000/LConn3 -- _CN_66098469_500000_CN216480979/RConn3
  _CN_170589736_500000_CN_161870227_500000/RConn1 -- T_170589736_500000_東近江/LConn1 -- _CN_170589736_500000_CN_170568495_500000/LConn1
  _CN_170589736_500000_CN_161870227_500000/RConn2 -- T_170589736_500000_東近江/LConn2 -- _CN_170589736_500000_CN_170568495_500000/LConn2
  _CN_170589736_500000_CN_161870227_500000/RConn3 -- T_170589736_500000_東近江/LConn3 -- _CN_170589736_500000_CN_170568495_500000/LConn3
  _CN_170589736_500000_CN_170568495_500000/RConn1 -- T_170568495_500000_三重開閉所/LConn1 -- _CN_170537514_500000_CN_170568495_500000/LConn1 -- _CN_170366035_500000_CN_170568495_500000/LConn1
  _CN_170589736_500000_CN_170568495_500000/RConn2 -- T_170568495_500000_三重開閉所/LConn2 -- _CN_170537514_500000_CN_170568495_500000/LConn2 -- _CN_170366035_500000_CN_170568495_500000/LConn2
  _CN_170589736_500000_CN_170568495_500000/RConn3 -- T_170568495_500000_三重開閉所/LConn3 -- _CN_170537514_500000_CN_170568495_500000/LConn3 -- _CN_170366035_500000_CN_170568495_500000/LConn3
  _CN_170537514_500000_CN_161946849_500000/LConn1 -- T_170537514_500000_/LConn1 -- _CN_170537514_500000_CN_170568495_500000/RConn1
  _CN_170537514_500000_CN_161946849_500000/LConn2 -- T_170537514_500000_/LConn2 -- _CN_170537514_500000_CN_170568495_500000/RConn2
  _CN_170537514_500000_CN_161946849_500000/LConn3 -- T_170537514_500000_/LConn3 -- _CN_170537514_500000_CN_170568495_500000/RConn3
  _CN_170537514_500000_CN_161946849_500000/RConn1 -- T_161946849_500000;275000_北部変電所/LConn1 -- _CN_169122898_500000_CN_161946849_500000/LConn1 -- _CN_170366035_500000_CN_161946849_500000/LConn1
  _CN_170537514_500000_CN_161946849_500000/RConn2 -- T_161946849_500000;275000_北部変電所/LConn2 -- _CN_169122898_500000_CN_161946849_500000/LConn2 -- _CN_170366035_500000_CN_161946849_500000/LConn2
  _CN_170537514_500000_CN_161946849_500000/RConn3 -- T_161946849_500000;275000_北部変電所/LConn3 -- _CN_169122898_500000_CN_161946849_500000/LConn3 -- _CN_170366035_500000_CN_161946849_500000/LConn3
  T_192745005_275000_丸山変電所_(Maruyama_Hendensho)/LConn1 -- 丸山幹線_(Maruyama_Kansen)_CN_192745005_275000_CN_161946848_275000/LConn1
  T_192745005_275000_丸山変電所_(Maruyama_Hendensho)/LConn2 -- 丸山幹線_(Maruyama_Kansen)_CN_192745005_275000_CN_161946848_275000/LConn2
  T_192745005_275000_丸山変電所_(Maruyama_Hendensho)/LConn3 -- 丸山幹線_(Maruyama_Kansen)_CN_192745005_275000_CN_161946848_275000/LConn3
  丸山幹線_(Maruyama_Kansen)_CN_192745005_275000_CN_161946848_275000/RConn1 -- T_161946848_275000_関開閉所_(Seki)/LConn1 -- _CN_161946848_275000_CN_190734269_275000/LConn1
  丸山幹線_(Maruyama_Kansen)_CN_192745005_275000_CN_161946848_275000/RConn2 -- T_161946848_275000_関開閉所_(Seki)/LConn2 -- _CN_161946848_275000_CN_190734269_275000/LConn2
  丸山幹線_(Maruyama_Kansen)_CN_192745005_275000_CN_161946848_275000/RConn3 -- T_161946848_275000_関開閉所_(Seki)/LConn3 -- _CN_161946848_275000_CN_190734269_275000/LConn3
  _CN_108199478_275000_CN_109834508_275000/LConn1 -- T_108199478_275000_南大阪変電所_(Minamiōsaka_Hendensho)/LConn1 -- 泉南東大阪線_(Sennan_Higashiōsaka_sen)_CN_108199478_275000_CN_158522649_275000/LConn1
  _CN_108199478_275000_CN_109834508_275000/LConn2 -- T_108199478_275000_南大阪変電所_(Minamiōsaka_Hendensho)/LConn2 -- 泉南東大阪線_(Sennan_Higashiōsaka_sen)_CN_108199478_275000_CN_158522649_275000/LConn2
  _CN_108199478_275000_CN_109834508_275000/LConn3 -- T_108199478_275000_南大阪変電所_(Minamiōsaka_Hendensho)/LConn3 -- 泉南東大阪線_(Sennan_Higashiōsaka_sen)_CN_108199478_275000_CN_158522649_275000/LConn3
  _CN_108199478_275000_CN_109834508_275000/RConn1 -- T_109834508_275000_金剛開閉所_(Kongō_Kaiheisho)/LConn1 -- 北葛城線_(Kita_Katsuragi_Sen)_CN_160374974_275000_CN_109834508_275000/LConn1 -- 金剛線_(Kongō_sen)_CN_109834508_275000_CN_291678103_275000/LConn1
  _CN_108199478_275000_CN_109834508_275000/RConn2 -- T_109834508_275000_金剛開閉所_(Kongō_Kaiheisho)/LConn2 -- 北葛城線_(Kita_Katsuragi_Sen)_CN_160374974_275000_CN_109834508_275000/LConn2 -- 金剛線_(Kongō_sen)_CN_109834508_275000_CN_291678103_275000/LConn2
  _CN_108199478_275000_CN_109834508_275000/RConn3 -- T_109834508_275000_金剛開閉所_(Kongō_Kaiheisho)/LConn3 -- 北葛城線_(Kita_Katsuragi_Sen)_CN_160374974_275000_CN_109834508_275000/LConn3 -- 金剛線_(Kongō_sen)_CN_109834508_275000_CN_291678103_275000/LConn3
  T_158522649_275000_東大阪変電所/LConn1 -- 泉南東大阪線_(Sennan_Higashiōsaka_sen)_CN_108199478_275000_CN_158522649_275000/RConn1
  T_158522649_275000_東大阪変電所/LConn2 -- 泉南東大阪線_(Sennan_Higashiōsaka_sen)_CN_108199478_275000_CN_158522649_275000/RConn2
  T_158522649_275000_東大阪変電所/LConn3 -- 泉南東大阪線_(Sennan_Higashiōsaka_sen)_CN_108199478_275000_CN_158522649_275000/RConn3
  T_315614776_275000_/LConn1 -- _CN_315614776_275000_CN_315614783_275000/LConn1
  T_315614776_275000_/LConn2 -- _CN_315614776_275000_CN_315614783_275000/LConn2
  T_315614776_275000_/LConn3 -- _CN_315614776_275000_CN_315614783_275000/LConn3
  T_315614783_275000_/LConn1 -- _CN_315614776_275000_CN_315614783_275000/RConn1
  T_315614783_275000_/LConn2 -- _CN_315614776_275000_CN_315614783_275000/RConn2
  T_315614783_275000_/LConn3 -- _CN_315614776_275000_CN_315614783_275000/RConn3
  T_316566585_275000_/LConn1 -- _CN_316566585_275000_CN_174636874_275000/LConn1
  T_316566585_275000_/LConn2 -- _CN_316566585_275000_CN_174636874_275000/LConn2
  T_316566585_275000_/LConn3 -- _CN_316566585_275000_CN_174636874_275000/LConn3
  _CN_316566585_275000_CN_174636874_275000/RConn1 -- T_174636874_275000_岩手変電所/LConn1 -- _CN_316566588_275000_CN_174636874_275000/LConn1
  _CN_316566585_275000_CN_174636874_275000/RConn2 -- T_174636874_275000_岩手変電所/LConn2 -- _CN_316566588_275000_CN_174636874_275000/LConn2
  _CN_316566585_275000_CN_174636874_275000/RConn3 -- T_174636874_275000_岩手変電所/LConn3 -- _CN_316566588_275000_CN_174636874_275000/LConn3
  _CN_316566588_275000_CN_316581632_275000/LConn1 -- T_316566588_275000_/LConn1 -- _CN_316566588_275000_CN_308348224_275000/LConn1 -- _CN_316566588_275000_CN_174636874_275000/RConn1
  _CN_316566588_275000_CN_316581632_275000/LConn2 -- T_316566588_275000_/LConn2 -- _CN_316566588_275000_CN_308348224_275000/LConn2 -- _CN_316566588_275000_CN_174636874_275000/RConn2
  _CN_316566588_275000_CN_316581632_275000/LConn3 -- T_316566588_275000_/LConn3 -- _CN_316566588_275000_CN_308348224_275000/LConn3 -- _CN_316566588_275000_CN_174636874_275000/RConn3
  T_316581632_275000_/LConn1 -- _CN_316566588_275000_CN_316581632_275000/RConn1
  T_316581632_275000_/LConn2 -- _CN_316566588_275000_CN_316581632_275000/RConn2
  T_316581632_275000_/LConn3 -- _CN_316566588_275000_CN_316581632_275000/RConn3
  T_308348224_275000_新庄変電所/LConn1 -- _CN_316566588_275000_CN_308348224_275000/RConn1
  T_308348224_275000_新庄変電所/LConn2 -- _CN_316566588_275000_CN_308348224_275000/RConn2
  T_308348224_275000_新庄変電所/LConn3 -- _CN_316566588_275000_CN_308348224_275000/RConn3
  T_116559939_500000_/LConn1 -- 駿遠幹線_CN_116559939_500000_CN_210090094_500000/LConn1
  T_116559939_500000_/LConn2 -- 駿遠幹線_CN_116559939_500000_CN_210090094_500000/LConn2
  T_116559939_500000_/LConn3 -- 駿遠幹線_CN_116559939_500000_CN_210090094_500000/LConn3
  T_210090094_500000_駿遠変電所/LConn1 -- 駿遠幹線_CN_116559939_500000_CN_210090094_500000/RConn1
  T_210090094_500000_駿遠変電所/LConn2 -- 駿遠幹線_CN_116559939_500000_CN_210090094_500000/RConn2
  T_210090094_500000_駿遠変電所/LConn3 -- 駿遠幹線_CN_116559939_500000_CN_210090094_500000/RConn3
  _CN_103818820_275000_CN_318218831_275000/LConn1 -- T_103818820_275000_仙台変電所/LConn1 -- _CN_103818820_275000_CN_250430935_275000/LConn1
  _CN_103818820_275000_CN_318218831_275000/LConn2 -- T_103818820_275000_仙台変電所/LConn2 -- _CN_103818820_275000_CN_250430935_275000/LConn2
  _CN_103818820_275000_CN_318218831_275000/LConn3 -- T_103818820_275000_仙台変電所/LConn3 -- _CN_103818820_275000_CN_250430935_275000/LConn3
  _CN_103818820_275000_CN_318218831_275000/RConn1 -- T_318218831_275000_/LConn1 -- _CN_318218831_275000_CN_169993955_275000/LConn1 -- _CN_318218831_275000_CN_319300956_275000/LConn1 -- _CN_318218831_275000_CN_170016148_275000/LConn1
  _CN_103818820_275000_CN_318218831_275000/RConn2 -- T_318218831_275000_/LConn2 -- _CN_318218831_275000_CN_169993955_275000/LConn2 -- _CN_318218831_275000_CN_319300956_275000/LConn2 -- _CN_318218831_275000_CN_170016148_275000/LConn2
  _CN_103818820_275000_CN_318218831_275000/RConn3 -- T_318218831_275000_/LConn3 -- _CN_318218831_275000_CN_169993955_275000/LConn3 -- _CN_318218831_275000_CN_319300956_275000/LConn3 -- _CN_318218831_275000_CN_170016148_275000/LConn3
  _CN_103818820_275000_CN_250430935_275000/RConn1 -- T_250430935_275000_米沢変電所_(Yonezawa_Hendensho)/LConn1 -- _CN_250430935_275000_CN_107262429_275000/LConn1 -- _CN_169993955_275000_CN_250430935_275000/LConn1 -- _CN_250430935_275000_CN354115662/LConn1
  _CN_103818820_275000_CN_250430935_275000/RConn2 -- T_250430935_275000_米沢変電所_(Yonezawa_Hendensho)/LConn2 -- _CN_250430935_275000_CN_107262429_275000/LConn2 -- _CN_169993955_275000_CN_250430935_275000/LConn2 -- _CN_250430935_275000_CN354115662/LConn2
  _CN_103818820_275000_CN_250430935_275000/RConn3 -- T_250430935_275000_米沢変電所_(Yonezawa_Hendensho)/LConn3 -- _CN_250430935_275000_CN_107262429_275000/LConn3 -- _CN_169993955_275000_CN_250430935_275000/LConn3 -- _CN_250430935_275000_CN354115662/LConn3
  T_172601929_500000;220000_/LConn1 -- _CN_172601929_500000_CN172644773/LConn1
  T_172601929_500000;220000_/LConn2 -- _CN_172601929_500000_CN172644773/LConn2
  T_172601929_500000;220000_/LConn3 -- _CN_172601929_500000_CN172644773/LConn3
  G_172644773_玄海原子力発電所/RConn1 -- _CN_172601929_500000_CN172644773/RConn1
  G_172644773_玄海原子力発電所/RConn2 -- _CN_172601929_500000_CN172644773/RConn2
  G_172644773_玄海原子力発電所/RConn3 -- _CN_172601929_500000_CN172644773/RConn3
  _CN_318218831_275000_CN_169993955_275000/RConn1 -- T_169993955_275000_新潟変電所/LConn1 -- _CN_169993955_275000_CN_250430935_275000/RConn1
  _CN_318218831_275000_CN_169993955_275000/RConn2 -- T_169993955_275000_新潟変電所/LConn2 -- _CN_169993955_275000_CN_250430935_275000/RConn2
  _CN_318218831_275000_CN_169993955_275000/RConn3 -- T_169993955_275000_新潟変電所/LConn3 -- _CN_169993955_275000_CN_250430935_275000/RConn3
  T_319300956_275000_中越変電所/LConn1 -- _CN_318218831_275000_CN_319300956_275000/RConn1
  T_319300956_275000_中越変電所/LConn2 -- _CN_318218831_275000_CN_319300956_275000/RConn2
  T_319300956_275000_中越変電所/LConn3 -- _CN_318218831_275000_CN_319300956_275000/RConn3
  T_170016148_275000_北新潟変電所/LConn1 -- _CN_318218831_275000_CN_170016148_275000/RConn1
  T_170016148_275000_北新潟変電所/LConn2 -- _CN_318218831_275000_CN_170016148_275000/RConn2
  T_170016148_275000_北新潟変電所/LConn3 -- _CN_318218831_275000_CN_170016148_275000/RConn3
  _CN_158064651_275000_CN_232998815_275000/LConn1 -- T_158064651_275000_田子倉発電所/LConn1 -- _CN_158064651_275000_CN319098734/LConn1
  _CN_158064651_275000_CN_232998815_275000/LConn2 -- T_158064651_275000_田子倉発電所/LConn2 -- _CN_158064651_275000_CN319098734/LConn2
  _CN_158064651_275000_CN_232998815_275000/LConn3 -- T_158064651_275000_田子倉発電所/LConn3 -- _CN_158064651_275000_CN319098734/LConn3
  _CN_158064651_275000_CN_232998815_275000/RConn1 -- T_232998815_275000_/LConn1 -- _CN_232998815_275000_CN233174201/LConn1
  _CN_158064651_275000_CN_232998815_275000/RConn2 -- T_232998815_275000_/LConn2 -- _CN_232998815_275000_CN233174201/LConn2
  _CN_158064651_275000_CN_232998815_275000/RConn3 -- T_232998815_275000_/LConn3 -- _CN_232998815_275000_CN233174201/LConn3
  _CN_158064651_275000_CN319098734/RConn1 -- G_319098734_信濃川水力発電所/RConn1 -- _CN_318302348_275000_CN319098734/LConn1
  _CN_158064651_275000_CN319098734/RConn2 -- G_319098734_信濃川水力発電所/RConn2 -- _CN_318302348_275000_CN319098734/LConn2
  _CN_158064651_275000_CN319098734/RConn3 -- G_319098734_信濃川水力発電所/RConn3 -- _CN_318302348_275000_CN319098734/LConn3
  _CN_169122898_500000_CN_161946849_500000/RConn1 -- T_169122898_500000_東部変電所/LConn1 -- _CN_169122898_500000_CN_142662111_500000/LConn1 -- _CN_169122898_500000_CN_170247312_500000/LConn1
  _CN_169122898_500000_CN_161946849_500000/RConn2 -- T_169122898_500000_東部変電所/LConn2 -- _CN_169122898_500000_CN_142662111_500000/LConn2 -- _CN_169122898_500000_CN_170247312_500000/LConn2
  _CN_169122898_500000_CN_161946849_500000/RConn3 -- T_169122898_500000_東部変電所/LConn3 -- _CN_169122898_500000_CN_142662111_500000/LConn3 -- _CN_169122898_500000_CN_170247312_500000/LConn3
  T_170247312_500000_新三河/LConn1 -- _CN_169122898_500000_CN_170247312_500000/RConn1
  T_170247312_500000_新三河/LConn2 -- _CN_169122898_500000_CN_170247312_500000/RConn2
  T_170247312_500000_新三河/LConn3 -- _CN_169122898_500000_CN_170247312_500000/RConn3
  _CN_169122898_500000_CN_142662111_500000/RConn1 -- T_142662111_500000_中部電力㈱豊根開閉所/LConn1 -- 南信幹線_CN_209429410_500000_CN_142662111_500000/LConn1 -- 豊根幹線_CN_170850727_500000_CN_142662111_500000/LConn1
  _CN_169122898_500000_CN_142662111_500000/RConn2 -- T_142662111_500000_中部電力㈱豊根開閉所/LConn2 -- 南信幹線_CN_209429410_500000_CN_142662111_500000/LConn2 -- 豊根幹線_CN_170850727_500000_CN_142662111_500000/LConn2
  _CN_169122898_500000_CN_142662111_500000/RConn3 -- T_142662111_500000_中部電力㈱豊根開閉所/LConn3 -- 南信幹線_CN_209429410_500000_CN_142662111_500000/LConn3 -- 豊根幹線_CN_170850727_500000_CN_142662111_500000/LConn3
  _CN_170366035_500000_CN_170568495_500000/RConn1 -- T_170366035_500000_/LConn1 -- _CN_170366035_500000_CN_170850727_500000/LConn1 -- _CN_170366035_500000_CN_161946849_500000/RConn1
  _CN_170366035_500000_CN_170568495_500000/RConn2 -- T_170366035_500000_/LConn2 -- _CN_170366035_500000_CN_170850727_500000/LConn2 -- _CN_170366035_500000_CN_161946849_500000/RConn2
  _CN_170366035_500000_CN_170568495_500000/RConn3 -- T_170366035_500000_/LConn3 -- _CN_170366035_500000_CN_170850727_500000/LConn3 -- _CN_170366035_500000_CN_161946849_500000/RConn3
  _CN_170366035_500000_CN_170850727_500000/RConn1 -- T_170850727_500000_愛知変電所/LConn1 -- 豊根幹線_CN_170850727_500000_CN_142662111_500000/RConn1
  _CN_170366035_500000_CN_170850727_500000/RConn2 -- T_170850727_500000_愛知変電所/LConn2 -- 豊根幹線_CN_170850727_500000_CN_142662111_500000/RConn2
  _CN_170366035_500000_CN_170850727_500000/RConn3 -- T_170850727_500000_愛知変電所/LConn3 -- 豊根幹線_CN_170850727_500000_CN_142662111_500000/RConn3
  T_170366036_275000_東豊田変電所/LConn1 -- _CN_170366036_275000_CN_170247359_275000/LConn1
  T_170366036_275000_東豊田変電所/LConn2 -- _CN_170366036_275000_CN_170247359_275000/LConn2
  T_170366036_275000_東豊田変電所/LConn3 -- _CN_170366036_275000_CN_170247359_275000/LConn3
  _CN_170366036_275000_CN_170247359_275000/RConn1 -- T_170247359_275000_/LConn1 -- _CN_170247314_275000_CN_170247359_275000/LConn1
  _CN_170366036_275000_CN_170247359_275000/RConn2 -- T_170247359_275000_/LConn2 -- _CN_170247314_275000_CN_170247359_275000/LConn2
  _CN_170366036_275000_CN_170247359_275000/RConn3 -- T_170247359_275000_/LConn3 -- _CN_170247314_275000_CN_170247359_275000/LConn3
  _CN_170366038_275000_CN_161946849_275000/LConn1 -- T_170366038_275000_/LConn1 -- _CN_170366038_275000_CN_169121278_275000/RConn1
  _CN_170366038_275000_CN_161946849_275000/LConn2 -- T_170366038_275000_/LConn2 -- _CN_170366038_275000_CN_169121278_275000/RConn2
  _CN_170366038_275000_CN_161946849_275000/LConn3 -- T_170366038_275000_/LConn3 -- _CN_170366038_275000_CN_169121278_275000/RConn3
  _CN_170366038_275000_CN_161946849_275000/RConn1 -- T_161946849_500000;275000_北部変電所/RConn1 -- _CN_161946849_275000_CN_161948515_275000/LConn1 -- _CN_161946849_275000_CN210658603/LConn1 -- L_161946849/LConn1
  _CN_170366038_275000_CN_161946849_275000/RConn2 -- T_161946849_500000;275000_北部変電所/RConn2 -- _CN_161946849_275000_CN_161948515_275000/LConn2 -- _CN_161946849_275000_CN210658603/LConn2 -- L_161946849/LConn2
  _CN_170366038_275000_CN_161946849_275000/RConn3 -- T_161946849_500000;275000_北部変電所/RConn3 -- _CN_161946849_275000_CN_161948515_275000/LConn3 -- _CN_161946849_275000_CN210658603/LConn3 -- L_161946849/LConn3
  _CN_242103481_500000_CN_241828221_500000/LConn1 -- T_242103481_500000_日野変電所/LConn1 -- _CN_242103481_500000_CN_317416612_500000/RConn1 -- _CN_242103481_500000_CN_317511904_500000/LConn1
  _CN_242103481_500000_CN_241828221_500000/LConn2 -- T_242103481_500000_日野変電所/LConn2 -- _CN_242103481_500000_CN_317416612_500000/RConn2 -- _CN_242103481_500000_CN_317511904_500000/LConn2
  _CN_242103481_500000_CN_241828221_500000/LConn3 -- T_242103481_500000_日野変電所/LConn3 -- _CN_242103481_500000_CN_317416612_500000/RConn3 -- _CN_242103481_500000_CN_317511904_500000/LConn3
  _CN_242103481_500000_CN_241828221_500000/RConn1 -- T_241828221_500000_新岡山変電所_(Shin_Okayama_Hendensho)/LConn1 -- _CN_241828221_500000_CN_241822623_500000/LConn1 -- _CN_170974371_500000_CN_241828221_500000/RConn1
  _CN_242103481_500000_CN_241828221_500000/RConn2 -- T_241828221_500000_新岡山変電所_(Shin_Okayama_Hendensho)/LConn2 -- _CN_241828221_500000_CN_241822623_500000/LConn2 -- _CN_170974371_500000_CN_241828221_500000/RConn2
  _CN_242103481_500000_CN_241828221_500000/RConn3 -- T_241828221_500000_新岡山変電所_(Shin_Okayama_Hendensho)/LConn3 -- _CN_241828221_500000_CN_241822623_500000/LConn3 -- _CN_170974371_500000_CN_241828221_500000/RConn3
  T_317511904_500000_北松江変電所/LConn1 -- _CN_242103481_500000_CN_317511904_500000/RConn1
  T_317511904_500000_北松江変電所/LConn2 -- _CN_242103481_500000_CN_317511904_500000/RConn2
  T_317511904_500000_北松江変電所/LConn3 -- _CN_242103481_500000_CN_317511904_500000/RConn3
  _CN_241956440_275000_CN214992492/LConn1 -- T_241956440_275000_伊勢開閉所/LConn1 -- _CN_241956440_275000_CN_241923317_275000/LConn1 -- _CN_241956440_275000_CN_242532736_275000/LConn1 -- 伊勢幹線_CN_241956440_275000_CN_170793703_275000/LConn1
  _CN_241956440_275000_CN214992492/LConn2 -- T_241956440_275000_伊勢開閉所/LConn2 -- _CN_241956440_275000_CN_241923317_275000/LConn2 -- _CN_241956440_275000_CN_242532736_275000/LConn2 -- 伊勢幹線_CN_241956440_275000_CN_170793703_275000/LConn2
  _CN_241956440_275000_CN214992492/LConn3 -- T_241956440_275000_伊勢開閉所/LConn3 -- _CN_241956440_275000_CN_241923317_275000/LConn3 -- _CN_241956440_275000_CN_242532736_275000/LConn3 -- 伊勢幹線_CN_241956440_275000_CN_170793703_275000/LConn3
  G_214992492_/RConn1 -- _CN_241956440_275000_CN214992492/RConn1
  G_214992492_/RConn2 -- _CN_241956440_275000_CN214992492/RConn2
  G_214992492_/RConn3 -- _CN_241956440_275000_CN214992492/RConn3
  T_242532736_275000_/LConn1 -- _CN_241956440_275000_CN_242532736_275000/RConn1
  T_242532736_275000_/LConn2 -- _CN_241956440_275000_CN_242532736_275000/RConn2
  T_242532736_275000_/LConn3 -- _CN_241956440_275000_CN_242532736_275000/RConn3
  伊勢幹線_CN_241956440_275000_CN_170793703_275000/RConn1 -- T_170793703_275000_西尾張/LConn1 -- _CN_170793702_275000_CN_170793703_275000/LConn1
  伊勢幹線_CN_241956440_275000_CN_170793703_275000/RConn2 -- T_170793703_275000_西尾張/LConn2 -- _CN_170793702_275000_CN_170793703_275000/LConn2
  伊勢幹線_CN_241956440_275000_CN_170793703_275000/RConn3 -- T_170793703_275000_西尾張/LConn3 -- _CN_170793702_275000_CN_170793703_275000/LConn3
  T_241923317_275000_南勢変電所_(Nansei_Hendensho)/LConn1 -- _CN_241956440_275000_CN_241923317_275000/RConn1
  T_241923317_275000_南勢変電所_(Nansei_Hendensho)/LConn2 -- _CN_241956440_275000_CN_241923317_275000/RConn2
  T_241923317_275000_南勢変電所_(Nansei_Hendensho)/LConn3 -- _CN_241956440_275000_CN_241923317_275000/RConn3
  _CN_87682157_275000_CN_128581912_275000/LConn1 -- T_87682157_275000_南川越変電所_(Minamikawagoe_Hendensho)/LConn1 -- _CN_87682157_275000_CN_159491797_275000/LConn1
  _CN_87682157_275000_CN_128581912_275000/LConn2 -- T_87682157_275000_南川越変電所_(Minamikawagoe_Hendensho)/LConn2 -- _CN_87682157_275000_CN_159491797_275000/LConn2
  _CN_87682157_275000_CN_128581912_275000/LConn3 -- T_87682157_275000_南川越変電所_(Minamikawagoe_Hendensho)/LConn3 -- _CN_87682157_275000_CN_159491797_275000/LConn3
  _CN_87682157_275000_CN_128581912_275000/RConn1 -- T_128581912_500000;275000;66000_新坂戸変電所/RConn1 -- 東京中線_CN_128581912_275000_CN_133137636_275000/LConn1 -- L_128581912/LConn1
  _CN_87682157_275000_CN_128581912_275000/RConn2 -- T_128581912_500000;275000;66000_新坂戸変電所/RConn2 -- 東京中線_CN_128581912_275000_CN_133137636_275000/LConn2 -- L_128581912/LConn2
  _CN_87682157_275000_CN_128581912_275000/RConn3 -- T_128581912_500000;275000;66000_新坂戸変電所/RConn3 -- 東京中線_CN_128581912_275000_CN_133137636_275000/LConn3 -- L_128581912/LConn3
  T_159491797_275000_南狭山変電所_(Minamisayama_Hendensho)/LConn1 -- _CN_87682157_275000_CN_159491797_275000/RConn1
  T_159491797_275000_南狭山変電所_(Minamisayama_Hendensho)/LConn2 -- _CN_87682157_275000_CN_159491797_275000/RConn2
  T_159491797_275000_南狭山変電所_(Minamisayama_Hendensho)/LConn3 -- _CN_87682157_275000_CN_159491797_275000/RConn3
  T_105291887_275000_那珂変電所_(Naka_Hendensho)/LConn1 -- _CN_105291887_275000_CN103827577/LConn1
  T_105291887_275000_那珂変電所_(Naka_Hendensho)/LConn2 -- _CN_105291887_275000_CN103827577/LConn2
  T_105291887_275000_那珂変電所_(Naka_Hendensho)/LConn3 -- _CN_105291887_275000_CN103827577/LConn3
  G_103827577_/RConn1 -- _CN_105291887_275000_CN103827577/RConn1
  G_103827577_/RConn2 -- _CN_105291887_275000_CN103827577/RConn2
  G_103827577_/RConn3 -- _CN_105291887_275000_CN103827577/RConn3
  _CN_320438391_500000_CN_241822621_500000/LConn1 -- T_320438391_500000_/LConn1 -- _CN_320438391_500000_CN_169031921_500000/RConn1 -- _CN_320438391_500000_CN_110682956_500000/LConn1 -- _CN_320438391_500000_CN_320444665_500000/LConn1
  _CN_320438391_500000_CN_241822621_500000/LConn2 -- T_320438391_500000_/LConn2 -- _CN_320438391_500000_CN_169031921_500000/RConn2 -- _CN_320438391_500000_CN_110682956_500000/LConn2 -- _CN_320438391_500000_CN_320444665_500000/LConn2
  _CN_320438391_500000_CN_241822621_500000/LConn3 -- T_320438391_500000_/LConn3 -- _CN_320438391_500000_CN_169031921_500000/RConn3 -- _CN_320438391_500000_CN_110682956_500000/LConn3 -- _CN_320438391_500000_CN_320444665_500000/LConn3
  T_241822621_500000_/LConn1 -- _CN_320438391_500000_CN_241822621_500000/RConn1
  T_241822621_500000_/LConn2 -- _CN_320438391_500000_CN_241822621_500000/RConn2
  T_241822621_500000_/LConn3 -- _CN_320438391_500000_CN_241822621_500000/RConn3
  _CN_320438391_500000_CN_110682956_500000/RConn1 -- T_110682956_500000_猪名川変電所/LConn1 -- _CN_110682956_500000_CN_170605907_500000/LConn1
  _CN_320438391_500000_CN_110682956_500000/RConn2 -- T_110682956_500000_猪名川変電所/LConn2 -- _CN_110682956_500000_CN_170605907_500000/LConn2
  _CN_320438391_500000_CN_110682956_500000/RConn3 -- T_110682956_500000_猪名川変電所/LConn3 -- _CN_110682956_500000_CN_170605907_500000/LConn3
  T_320444665_500000_/LConn1 -- _CN_320438391_500000_CN_320444665_500000/RConn1
  T_320444665_500000_/LConn2 -- _CN_320438391_500000_CN_320444665_500000/RConn2
  T_320444665_500000_/LConn3 -- _CN_320438391_500000_CN_320444665_500000/RConn3
  T_179417733_275000_/LConn1 -- _CN_179417733_275000_CN180359744/LConn1
  T_179417733_275000_/LConn2 -- _CN_179417733_275000_CN180359744/LConn2
  T_179417733_275000_/LConn3 -- _CN_179417733_275000_CN180359744/LConn3
  G_180359744_知多火力発電所/RConn1 -- _CN_179417733_275000_CN180359744/RConn1
  G_180359744_知多火力発電所/RConn2 -- _CN_179417733_275000_CN180359744/RConn2
  G_180359744_知多火力発電所/RConn3 -- _CN_179417733_275000_CN180359744/RConn3
  T_315461259_500000_/LConn1 -- 富津火力線_CN_315461259_500000_CN_315461272_500000/LConn1
  T_315461259_500000_/LConn2 -- 富津火力線_CN_315461259_500000_CN_315461272_500000/LConn2
  T_315461259_500000_/LConn3 -- 富津火力線_CN_315461259_500000_CN_315461272_500000/LConn3
  富津火力線_CN_315461259_500000_CN_315461272_500000/RConn1 -- T_315461272_500000_新木更津変電所/LConn1 -- _CN_315461272_500000_CN_105298089_500000/LConn1
  富津火力線_CN_315461259_500000_CN_315461272_500000/RConn2 -- T_315461272_500000_新木更津変電所/LConn2 -- _CN_315461272_500000_CN_105298089_500000/LConn2
  富津火力線_CN_315461259_500000_CN_315461272_500000/RConn3 -- T_315461272_500000_新木更津変電所/LConn3 -- _CN_315461272_500000_CN_105298089_500000/LConn3
  T_170247308_275000_三河変電所/LConn1 -- 湖西三河線_CN_170247308_275000_CN_170260165_275000/LConn1
  T_170247308_275000_三河変電所/LConn2 -- 湖西三河線_CN_170247308_275000_CN_170260165_275000/LConn2
  T_170247308_275000_三河変電所/LConn3 -- 湖西三河線_CN_170247308_275000_CN_170260165_275000/LConn3
  T_170260165_275000_中部電力湖西変電所/LConn1 -- 湖西三河線_CN_170247308_275000_CN_170260165_275000/RConn1
  T_170260165_275000_中部電力湖西変電所/LConn2 -- 湖西三河線_CN_170247308_275000_CN_170260165_275000/RConn2
  T_170260165_275000_中部電力湖西変電所/LConn3 -- 湖西三河線_CN_170247308_275000_CN_170260165_275000/RConn3
  東京中線_CN_128581912_275000_CN_133137636_275000/RConn1 -- T_133137636_275000_北東京変電所_(Kita_Tōkyō_Hendensho)/LConn1 -- 西越谷線_(Nishi_Koshigaya_Sen)_CN_153521822_275000_CN_133137636_275000/LConn1
  東京中線_CN_128581912_275000_CN_133137636_275000/RConn2 -- T_133137636_275000_北東京変電所_(Kita_Tōkyō_Hendensho)/LConn2 -- 西越谷線_(Nishi_Koshigaya_Sen)_CN_153521822_275000_CN_133137636_275000/LConn2
  東京中線_CN_128581912_275000_CN_133137636_275000/RConn3 -- T_133137636_275000_北東京変電所_(Kita_Tōkyō_Hendensho)/LConn3 -- 西越谷線_(Nishi_Koshigaya_Sen)_CN_153521822_275000_CN_133137636_275000/LConn3
  T_128581912_500000;275000;66000_新坂戸変電所/LConn1 -- 新坂戸線_CN_128581912_500000_CN_133641619_500000/LConn1
  T_128581912_500000;275000;66000_新坂戸変電所/LConn2 -- 新坂戸線_CN_128581912_500000_CN_133641619_500000/LConn2
  T_128581912_500000;275000;66000_新坂戸変電所/LConn3 -- 新坂戸線_CN_128581912_500000_CN_133641619_500000/LConn3
  新坂戸線_CN_128581912_500000_CN_133641619_500000/RConn1 -- T_133641619_500000_新所沢変電所_(Shin_Tokorozawa_Hendensho)/LConn1 -- 新所沢線_(Shin_Tokorozawa_Sen)_CN_133641619_500000_CN_145079972_500000/RConn1 -- 新古河線_(Shin_Koga_Sen)_CN_133135172_500000_CN_133641619_500000/LConn1
  新坂戸線_CN_128581912_500000_CN_133641619_500000/RConn2 -- T_133641619_500000_新所沢変電所_(Shin_Tokorozawa_Hendensho)/LConn2 -- 新所沢線_(Shin_Tokorozawa_Sen)_CN_133641619_500000_CN_145079972_500000/RConn2 -- 新古河線_(Shin_Koga_Sen)_CN_133135172_500000_CN_133641619_500000/LConn2
  新坂戸線_CN_128581912_500000_CN_133641619_500000/RConn3 -- T_133641619_500000_新所沢変電所_(Shin_Tokorozawa_Hendensho)/LConn3 -- 新所沢線_(Shin_Tokorozawa_Sen)_CN_133641619_500000_CN_145079972_500000/RConn3 -- 新古河線_(Shin_Koga_Sen)_CN_133135172_500000_CN_133641619_500000/LConn3
  T_170247314_275000_額田開閉所/LConn1 -- _CN_170247314_275000_CN_170247359_275000/RConn1
  T_170247314_275000_額田開閉所/LConn2 -- _CN_170247314_275000_CN_170247359_275000/RConn2
  T_170247314_275000_額田開閉所/LConn3 -- _CN_170247314_275000_CN_170247359_275000/RConn3
  _CN_315608215_500000_CN_169249243_500000/LConn1 -- T_315608215_500000_/LConn1 -- _CN_315608215_500000_CN_169249247_500000/LConn1 -- 志賀中能登線_CN_315608215_500000_CN255763556/LConn1
  _CN_315608215_500000_CN_169249243_500000/LConn2 -- T_315608215_500000_/LConn2 -- _CN_315608215_500000_CN_169249247_500000/LConn2 -- 志賀中能登線_CN_315608215_500000_CN255763556/LConn2
  _CN_315608215_500000_CN_169249243_500000/LConn3 -- T_315608215_500000_/LConn3 -- _CN_315608215_500000_CN_169249247_500000/LConn3 -- 志賀中能登線_CN_315608215_500000_CN255763556/LConn3
  _CN_315608215_500000_CN_169249243_500000/RConn1 -- T_169249243_500000_南福光変電所/LConn1 -- 加賀福光線_CN_169249243_500000_CN_169249247_500000/LConn1
  _CN_315608215_500000_CN_169249243_500000/RConn2 -- T_169249243_500000_南福光変電所/LConn2 -- 加賀福光線_CN_169249243_500000_CN_169249247_500000/LConn2
  _CN_315608215_500000_CN_169249243_500000/RConn3 -- T_169249243_500000_南福光変電所/LConn3 -- 加賀福光線_CN_169249243_500000_CN_169249247_500000/LConn3
  _CN_315608215_500000_CN_169249247_500000/RConn1 -- T_169249247_500000_加賀変電所/LConn1 -- 加賀福光線_CN_169249243_500000_CN_169249247_500000/RConn1
  _CN_315608215_500000_CN_169249247_500000/RConn2 -- T_169249247_500000_加賀変電所/LConn2 -- 加賀福光線_CN_169249243_500000_CN_169249247_500000/RConn2
  _CN_315608215_500000_CN_169249247_500000/RConn3 -- T_169249247_500000_加賀変電所/LConn3 -- 加賀福光線_CN_169249243_500000_CN_169249247_500000/RConn3
  G_255763556_志賀原子力発電所/RConn1 -- 志賀中能登線_CN_315608215_500000_CN255763556/RConn1
  G_255763556_志賀原子力発電所/RConn2 -- 志賀中能登線_CN_315608215_500000_CN255763556/RConn2
  G_255763556_志賀原子力発電所/RConn3 -- 志賀中能登線_CN_315608215_500000_CN255763556/RConn3
  _CN_315461272_500000_CN_105298089_500000/RConn1 -- T_105298089_500000_新佐原変電所/LConn1 -- _CN_105298089_500000_CN_168727982_500000/LConn1 -- _CN_105298089_500000_CN_132913106_500000/LConn1
  _CN_315461272_500000_CN_105298089_500000/RConn2 -- T_105298089_500000_新佐原変電所/LConn2 -- _CN_105298089_500000_CN_168727982_500000/LConn2 -- _CN_105298089_500000_CN_132913106_500000/LConn2
  _CN_315461272_500000_CN_105298089_500000/RConn3 -- T_105298089_500000_新佐原変電所/LConn3 -- _CN_105298089_500000_CN_168727982_500000/LConn3 -- _CN_105298089_500000_CN_132913106_500000/LConn3
  T_153521822_275000_西越谷変電所_(Nishi_Koshigaya_Hendensho)/LConn1 -- 西越谷線_(Nishi_Koshigaya_Sen)_CN_153521822_275000_CN_133137636_275000/RConn1
  T_153521822_275000_西越谷変電所_(Nishi_Koshigaya_Hendensho)/LConn2 -- 西越谷線_(Nishi_Koshigaya_Sen)_CN_153521822_275000_CN_133137636_275000/RConn2
  T_153521822_275000_西越谷変電所_(Nishi_Koshigaya_Hendensho)/LConn3 -- 西越谷線_(Nishi_Koshigaya_Sen)_CN_153521822_275000_CN_133137636_275000/RConn3
  _CN_317416612_500000_CN_204258596_500000/RConn1 -- T_204258596_500000_/LConn1 -- _CN_242253500_500000_CN_204258596_500000/RConn1 -- 関門連系線_CN_204258596_500000_CN_187988970_500000/RConn1
  _CN_317416612_500000_CN_204258596_500000/RConn2 -- T_204258596_500000_/LConn2 -- _CN_242253500_500000_CN_204258596_500000/RConn2 -- 関門連系線_CN_204258596_500000_CN_187988970_500000/RConn2
  _CN_317416612_500000_CN_204258596_500000/RConn3 -- T_204258596_500000_/LConn3 -- _CN_242253500_500000_CN_204258596_500000/RConn3 -- 関門連系線_CN_204258596_500000_CN_187988970_500000/RConn3
  _CN_87538349_500000_CN_171066843_500000/LConn1 -- T_87538349_500000_讃岐変電所/LConn1 -- _CN_87538349_500000_CN_102958903_500000/LConn1
  _CN_87538349_500000_CN_171066843_500000/LConn2 -- T_87538349_500000_讃岐変電所/LConn2 -- _CN_87538349_500000_CN_102958903_500000/LConn2
  _CN_87538349_500000_CN_171066843_500000/LConn3 -- T_87538349_500000_讃岐変電所/LConn3 -- _CN_87538349_500000_CN_102958903_500000/LConn3
  T_171066843_500000_四国電力東予変電所/LConn1 -- _CN_87538349_500000_CN_171066843_500000/RConn1
  T_171066843_500000_四国電力東予変電所/LConn2 -- _CN_87538349_500000_CN_171066843_500000/RConn2
  T_171066843_500000_四国電力東予変電所/LConn3 -- _CN_87538349_500000_CN_171066843_500000/RConn3
  T_102958903_500000_/LConn1 -- _CN_87538349_500000_CN_102958903_500000/RConn1
  T_102958903_500000_/LConn2 -- _CN_87538349_500000_CN_102958903_500000/RConn2
  T_102958903_500000_/LConn3 -- _CN_87538349_500000_CN_102958903_500000/RConn3
  T_242253497_275000_姫路変電所_(Himeji_Hendensho)/LConn1 -- _CN_242253497_275000_CN_185032690_275000/LConn1
  T_242253497_275000_姫路変電所_(Himeji_Hendensho)/LConn2 -- _CN_242253497_275000_CN_185032690_275000/LConn2
  T_242253497_275000_姫路変電所_(Himeji_Hendensho)/LConn3 -- _CN_242253497_275000_CN_185032690_275000/LConn3
  _CN_242253497_275000_CN_185032690_275000/RConn1 -- T_185032690_275000_西神戸変電所/LConn1 -- _CN_185032690_275000_CN110340505/LConn1
  _CN_242253497_275000_CN_185032690_275000/RConn2 -- T_185032690_275000_西神戸変電所/LConn2 -- _CN_185032690_275000_CN110340505/LConn2
  _CN_242253497_275000_CN_185032690_275000/RConn3 -- T_185032690_275000_西神戸変電所/LConn3 -- _CN_185032690_275000_CN110340505/LConn3
  T_160374974_275000;77000_北葛城変電所_(Kita_Katsuragi_Hendensho)/LConn1 -- 北葛城線_(Kita_Katsuragi_Sen)_CN_160374974_275000_CN_109834508_275000/RConn1
  T_160374974_275000;77000_北葛城変電所_(Kita_Katsuragi_Hendensho)/LConn2 -- 北葛城線_(Kita_Katsuragi_Sen)_CN_160374974_275000_CN_109834508_275000/RConn2
  T_160374974_275000;77000_北葛城変電所_(Kita_Katsuragi_Hendensho)/LConn3 -- 北葛城線_(Kita_Katsuragi_Sen)_CN_160374974_275000_CN_109834508_275000/RConn3
  T_302164679_275000_能代変電所/LConn1 -- _CN_302164679_275000_CN_316581637_275000/LConn1
  T_302164679_275000_能代変電所/LConn2 -- _CN_302164679_275000_CN_316581637_275000/LConn2
  T_302164679_275000_能代変電所/LConn3 -- _CN_302164679_275000_CN_316581637_275000/LConn3
  T_316581637_275000_青森変電所/LConn1 -- _CN_302164679_275000_CN_316581637_275000/RConn1
  T_316581637_275000_青森変電所/LConn2 -- _CN_302164679_275000_CN_316581637_275000/RConn2
  T_316581637_275000_青森変電所/LConn3 -- _CN_302164679_275000_CN_316581637_275000/RConn3
  T_216956620_500000_/LConn1 -- 小丸川幹線_CN_216956620_500000_CN216953915/LConn1
  T_216956620_500000_/LConn2 -- 小丸川幹線_CN_216956620_500000_CN216953915/LConn2
  T_216956620_500000_/LConn3 -- 小丸川幹線_CN_216956620_500000_CN216953915/LConn3
  G_216953915_/RConn1 -- 小丸川幹線_CN_216956620_500000_CN216953915/RConn1
  G_216953915_/RConn2 -- 小丸川幹線_CN_216956620_500000_CN216953915/RConn2
  G_216953915_/RConn3 -- 小丸川幹線_CN_216956620_500000_CN216953915/RConn3
  T_159191758_275000_北松本変電所/LConn1 -- _CN_159191758_275000_CN_211258348_275000/LConn1
  T_159191758_275000_北松本変電所/LConn2 -- _CN_159191758_275000_CN_211258348_275000/LConn2
  T_159191758_275000_北松本変電所/LConn3 -- _CN_159191758_275000_CN_211258348_275000/LConn3
  _CN_159191758_275000_CN_211258348_275000/RConn1 -- T_211258348_275000_東信変電所/LConn1 -- _CN_199544541_275000_CN_211258348_275000/LConn1
  _CN_159191758_275000_CN_211258348_275000/RConn2 -- T_211258348_275000_東信変電所/LConn2 -- _CN_199544541_275000_CN_211258348_275000/LConn2
  _CN_159191758_275000_CN_211258348_275000/RConn3 -- T_211258348_275000_東信変電所/LConn3 -- _CN_199544541_275000_CN_211258348_275000/LConn3
  T_169963227_500000_新榛名/LConn1 -- 新榛名線_CN_169963227_500000_CN_195615141_500000/LConn1
  T_169963227_500000_新榛名/LConn2 -- 新榛名線_CN_169963227_500000_CN_195615141_500000/LConn2
  T_169963227_500000_新榛名/LConn3 -- 新榛名線_CN_169963227_500000_CN_195615141_500000/LConn3
  新榛名線_CN_169963227_500000_CN_195615141_500000/RConn1 -- T_195615141_500000_/LConn1 -- _CN_195615141_500000_CN_145079972_500000/RConn1 -- _CN_195615141_500000_CN_315662839_500000/LConn1
  新榛名線_CN_169963227_500000_CN_195615141_500000/RConn2 -- T_195615141_500000_/LConn2 -- _CN_195615141_500000_CN_145079972_500000/RConn2 -- _CN_195615141_500000_CN_315662839_500000/LConn2
  新榛名線_CN_169963227_500000_CN_195615141_500000/RConn3 -- T_195615141_500000_/LConn3 -- _CN_195615141_500000_CN_145079972_500000/RConn3 -- _CN_195615141_500000_CN_315662839_500000/LConn3
  T_199544541_275000_新北信変電所/LConn1 -- _CN_199544541_275000_CN_211258348_275000/RConn1
  T_199544541_275000_新北信変電所/LConn2 -- _CN_199544541_275000_CN_211258348_275000/RConn2
  T_199544541_275000_新北信変電所/LConn3 -- _CN_199544541_275000_CN_211258348_275000/RConn3
  T_190734269_275000_/LConn1 -- _CN_161946848_275000_CN_190734269_275000/RConn1
  T_190734269_275000_/LConn2 -- _CN_161946848_275000_CN_190734269_275000/RConn2
  T_190734269_275000_/LConn3 -- _CN_161946848_275000_CN_190734269_275000/RConn3
  T_161948515_275000_西濃変電所_(Seinō_Hendensho)/LConn1 -- _CN_161946849_275000_CN_161948515_275000/RConn1
  T_161948515_275000_西濃変電所_(Seinō_Hendensho)/LConn2 -- _CN_161946849_275000_CN_161948515_275000/RConn2
  T_161948515_275000_西濃変電所_(Seinō_Hendensho)/LConn3 -- _CN_161946849_275000_CN_161948515_275000/RConn3
  G_210658603_高根第一水力発電所/RConn1 -- _CN_161946849_275000_CN210658603/RConn1
  G_210658603_高根第一水力発電所/RConn2 -- _CN_161946849_275000_CN210658603/RConn2
  G_210658603_高根第一水力発電所/RConn3 -- _CN_161946849_275000_CN210658603/RConn3
  _CN_170793702_275000_CN_170793703_275000/RConn1 -- T_170793702_275000_西名古屋/LConn1 -- _CN_170793702_275000_CN180359727/LConn1
  _CN_170793702_275000_CN_170793703_275000/RConn2 -- T_170793702_275000_西名古屋/LConn2 -- _CN_170793702_275000_CN180359727/LConn2
  _CN_170793702_275000_CN_170793703_275000/RConn3 -- T_170793702_275000_西名古屋/LConn3 -- _CN_170793702_275000_CN180359727/LConn3
  G_180359727_川越火力発電所/RConn1 -- _CN_170793702_275000_CN180359727/RConn1
  G_180359727_川越火力発電所/RConn2 -- _CN_170793702_275000_CN180359727/RConn2
  G_180359727_川越火力発電所/RConn3 -- _CN_170793702_275000_CN180359727/RConn3
  T_242103532_500000_/LConn1 -- _CN_242103532_500000_CN_241822623_500000/LConn1
  T_242103532_500000_/LConn2 -- _CN_242103532_500000_CN_241822623_500000/LConn2
  T_242103532_500000_/LConn3 -- _CN_242103532_500000_CN_241822623_500000/LConn3
  _CN_242103532_500000_CN_241822623_500000/RConn1 -- T_241822623_500000;220000;110000_/LConn1 -- _CN_241828221_500000_CN_241822623_500000/RConn1
  _CN_242103532_500000_CN_241822623_500000/RConn2 -- T_241822623_500000;220000;110000_/LConn2 -- _CN_241828221_500000_CN_241822623_500000/RConn2
  _CN_242103532_500000_CN_241822623_500000/RConn3 -- T_241822623_500000;220000;110000_/LConn3 -- _CN_241828221_500000_CN_241822623_500000/RConn3
  G_379474501_/RConn1 -- 東京南線3;4号線_CN_128364781_275000_CN379474501/RConn1
  G_379474501_/RConn2 -- 東京南線3;4号線_CN_128364781_275000_CN379474501/RConn2
  G_379474501_/RConn3 -- 東京南線3;4号線_CN_128364781_275000_CN379474501/RConn3
  京浜線1;2号線_CN_128364781_275000_CN_47110637_275000/RConn1 -- T_47110637_275000_西東京変電所/LConn1 -- 東京西線_CN_145080115_275000_CN_47110637_275000/LConn1
  京浜線1;2号線_CN_128364781_275000_CN_47110637_275000/RConn2 -- T_47110637_275000_西東京変電所/LConn2 -- 東京西線_CN_145080115_275000_CN_47110637_275000/LConn2
  京浜線1;2号線_CN_128364781_275000_CN_47110637_275000/RConn3 -- T_47110637_275000_西東京変電所/LConn3 -- 東京西線_CN_145080115_275000_CN_47110637_275000/LConn3
  T_104375141_275000_須賀川変電所_(Sukagawa_Hendensho)/LConn1 -- _CN_104375141_275000_CN_107262429_275000/LConn1
  T_104375141_275000_須賀川変電所_(Sukagawa_Hendensho)/LConn2 -- _CN_104375141_275000_CN_107262429_275000/LConn2
  T_104375141_275000_須賀川変電所_(Sukagawa_Hendensho)/LConn3 -- _CN_104375141_275000_CN_107262429_275000/LConn3
  _CN_104375141_275000_CN_107262429_275000/RConn1 -- T_107262429_275000_福島変電所/LConn1 -- _CN_316459359_275000_CN_107262429_275000/LConn1 -- _CN_250430935_275000_CN_107262429_275000/RConn1
  _CN_104375141_275000_CN_107262429_275000/RConn2 -- T_107262429_275000_福島変電所/LConn2 -- _CN_316459359_275000_CN_107262429_275000/LConn2 -- _CN_250430935_275000_CN_107262429_275000/RConn2
  _CN_104375141_275000_CN_107262429_275000/RConn3 -- T_107262429_275000_福島変電所/LConn3 -- _CN_316459359_275000_CN_107262429_275000/LConn3 -- _CN_250430935_275000_CN_107262429_275000/RConn3
  T_250540807_500000_東群馬変電所_(Higashi_Gunma_Substation)/LConn1 -- 東群馬幹線_CN_250540807_500000_CN_66098469_500000/RConn1
  T_250540807_500000_東群馬変電所_(Higashi_Gunma_Substation)/LConn2 -- 東群馬幹線_CN_250540807_500000_CN_66098469_500000/RConn2
  T_250540807_500000_東群馬変電所_(Higashi_Gunma_Substation)/LConn3 -- 東群馬幹線_CN_250540807_500000_CN_66098469_500000/RConn3
  G_354115662_沼沢発電所/RConn1 -- _CN_250430935_275000_CN354115662/RConn1
  G_354115662_沼沢発電所/RConn2 -- _CN_250430935_275000_CN354115662/RConn2
  G_354115662_沼沢発電所/RConn3 -- _CN_250430935_275000_CN354115662/RConn3
  T_291678103_275000_紀の川変電所_(Kinokawa_Hendensho)/LConn1 -- 金剛線_(Kongō_sen)_CN_109834508_275000_CN_291678103_275000/RConn1
  T_291678103_275000_紀の川変電所_(Kinokawa_Hendensho)/LConn2 -- 金剛線_(Kongō_sen)_CN_109834508_275000_CN_291678103_275000/RConn2
  T_291678103_275000_紀の川変電所_(Kinokawa_Hendensho)/LConn3 -- 金剛線_(Kongō_sen)_CN_109834508_275000_CN_291678103_275000/RConn3
  T_151379730_500000_房総変電所_(Bōsō_Hendensho)/LConn1 -- 房総線_CN_151379730_500000_CN_168727982_500000/LConn1
  T_151379730_500000_房総変電所_(Bōsō_Hendensho)/LConn2 -- 房総線_CN_151379730_500000_CN_168727982_500000/LConn2
  T_151379730_500000_房総変電所_(Bōsō_Hendensho)/LConn3 -- 房総線_CN_151379730_500000_CN_168727982_500000/LConn3
  房総線_CN_151379730_500000_CN_168727982_500000/RConn1 -- T_168727982_500000_新京葉変電所/LConn1 -- _CN_105298089_500000_CN_168727982_500000/RConn1 -- 新京葉線_CN_133135172_500000_CN_168727982_500000/LConn1
  房総線_CN_151379730_500000_CN_168727982_500000/RConn2 -- T_168727982_500000_新京葉変電所/LConn2 -- _CN_105298089_500000_CN_168727982_500000/RConn2 -- 新京葉線_CN_133135172_500000_CN_168727982_500000/LConn2
  房総線_CN_151379730_500000_CN_168727982_500000/RConn3 -- T_168727982_500000_新京葉変電所/LConn3 -- _CN_105298089_500000_CN_168727982_500000/RConn3 -- 新京葉線_CN_133135172_500000_CN_168727982_500000/LConn3
  T_215451416_500000;220000_九州電力南九州変電所/LConn1 -- _CN_215451416_500000_CN215429864/LConn1
  T_215451416_500000;220000_九州電力南九州変電所/LConn2 -- _CN_215451416_500000_CN215429864/LConn2
  T_215451416_500000;220000_九州電力南九州変電所/LConn3 -- _CN_215451416_500000_CN215429864/LConn3
  G_215429864_川内原子力発電所/RConn1 -- _CN_215451416_500000_CN215429864/RConn1
  G_215429864_川内原子力発電所/RConn2 -- _CN_215451416_500000_CN215429864/RConn2
  G_215429864_川内原子力発電所/RConn3 -- _CN_215451416_500000_CN215429864/RConn3
  T_325868333_275000_/LConn1 -- _CN_325868333_275000_CN_110682951_275000/LConn1
  T_325868333_275000_/LConn2 -- _CN_325868333_275000_CN_110682951_275000/LConn2
  T_325868333_275000_/LConn3 -- _CN_325868333_275000_CN_110682951_275000/LConn3
  _CN_325868333_275000_CN_110682951_275000/RConn1 -- T_110682951_275000_宝塚開閉所_(Takarazuka_Kaiheisho)/LConn1 -- _CN_110682951_275000_CN_110682955_275000/LConn1
  _CN_325868333_275000_CN_110682951_275000/RConn2 -- T_110682951_275000_宝塚開閉所_(Takarazuka_Kaiheisho)/LConn2 -- _CN_110682951_275000_CN_110682955_275000/LConn2
  _CN_325868333_275000_CN_110682951_275000/RConn3 -- T_110682951_275000_宝塚開閉所_(Takarazuka_Kaiheisho)/LConn3 -- _CN_110682951_275000_CN_110682955_275000/LConn3
  T_145080115_275000_/LConn1 -- 東京西線_CN_145080115_275000_CN_47110637_275000/RConn1
  T_145080115_275000_/LConn2 -- 東京西線_CN_145080115_275000_CN_47110637_275000/RConn2
  T_145080115_275000_/LConn3 -- 東京西線_CN_145080115_275000_CN_47110637_275000/RConn3
  新古河線_(Shin_Koga_Sen)_CN_133135172_500000_CN_133641619_500000/RConn1 -- T_133135172_500000_新古河変電所/LConn1 -- 新京葉線_CN_133135172_500000_CN_168727982_500000/RConn1 -- 新筑波線_(Shin_Tsukuba_Sen)_CN_133135172_500000_CN_132913106_500000/LConn1
  新古河線_(Shin_Koga_Sen)_CN_133135172_500000_CN_133641619_500000/RConn2 -- T_133135172_500000_新古河変電所/LConn2 -- 新京葉線_CN_133135172_500000_CN_168727982_500000/RConn2 -- 新筑波線_(Shin_Tsukuba_Sen)_CN_133135172_500000_CN_132913106_500000/LConn2
  新古河線_(Shin_Koga_Sen)_CN_133135172_500000_CN_133641619_500000/RConn3 -- T_133135172_500000_新古河変電所/LConn3 -- 新京葉線_CN_133135172_500000_CN_168727982_500000/RConn3 -- 新筑波線_(Shin_Tsukuba_Sen)_CN_133135172_500000_CN_132913106_500000/LConn3
  新筑波線_(Shin_Tsukuba_Sen)_CN_133135172_500000_CN_132913106_500000/RConn1 -- T_132913106_500000_新筑波変電所_(Shin_Tsukuba_Hendensho)/LConn1 -- _CN_105298089_500000_CN_132913106_500000/RConn1 -- _CN_132913106_500000_CN_104391636_500000/LConn1
  新筑波線_(Shin_Tsukuba_Sen)_CN_133135172_500000_CN_132913106_500000/RConn2 -- T_132913106_500000_新筑波変電所_(Shin_Tsukuba_Hendensho)/LConn2 -- _CN_105298089_500000_CN_132913106_500000/RConn2 -- _CN_132913106_500000_CN_104391636_500000/LConn2
  新筑波線_(Shin_Tsukuba_Sen)_CN_133135172_500000_CN_132913106_500000/RConn3 -- T_132913106_500000_新筑波変電所_(Shin_Tsukuba_Hendensho)/LConn3 -- _CN_105298089_500000_CN_132913106_500000/RConn3 -- _CN_132913106_500000_CN_104391636_500000/LConn3
  T_110682955_275000;154000;77000_伊丹変電所_(Itami_Hendensho)/LConn1 -- _CN_110682951_275000_CN_110682955_275000/RConn1
  T_110682955_275000;154000;77000_伊丹変電所_(Itami_Hendensho)/LConn2 -- _CN_110682951_275000_CN_110682955_275000/RConn2
  T_110682955_275000;154000;77000_伊丹変電所_(Itami_Hendensho)/LConn3 -- _CN_110682951_275000_CN_110682955_275000/RConn3
  T_318302348_275000_東上越変電所/LConn1 -- _CN_318302348_275000_CN319098734/RConn1
  T_318302348_275000_東上越変電所/LConn2 -- _CN_318302348_275000_CN319098734/RConn2
  T_318302348_275000_東上越変電所/LConn3 -- _CN_318302348_275000_CN319098734/RConn3
  T_170605907_500000_北摂変電所/LConn1 -- _CN_110682956_500000_CN_170605907_500000/RConn1
  T_170605907_500000_北摂変電所/LConn2 -- _CN_110682956_500000_CN_170605907_500000/RConn2
  T_170605907_500000_北摂変電所/LConn3 -- _CN_110682956_500000_CN_170605907_500000/RConn3
  T_185029969_500000;220000_/LConn1 -- _CN_185029969_500000_CN216798219/LConn1
  T_185029969_500000;220000_/LConn2 -- _CN_185029969_500000_CN216798219/LConn2
  T_185029969_500000;220000_/LConn3 -- _CN_185029969_500000_CN216798219/LConn3
  G_216798219_九州電力_松浦火力発電所/RConn1 -- _CN_185029969_500000_CN216798219/RConn1
  G_216798219_九州電力_松浦火力発電所/RConn2 -- _CN_185029969_500000_CN216798219/RConn2
  G_216798219_九州電力_松浦火力発電所/RConn3 -- _CN_185029969_500000_CN216798219/RConn3
  T_316459359_275000_/LConn1 -- _CN_316459359_275000_CN_107262429_275000/RConn1
  T_316459359_275000_/LConn2 -- _CN_316459359_275000_CN_107262429_275000/RConn2
  T_316459359_275000_/LConn3 -- _CN_316459359_275000_CN_107262429_275000/RConn3
  福島東幹線2_CN_106309481_500000_CN_104391636_500000/RConn1 -- T_104391636_500000_新いわき/LConn1 -- _CN_132913106_500000_CN_104391636_500000/RConn1
  福島東幹線2_CN_106309481_500000_CN_104391636_500000/RConn2 -- T_104391636_500000_新いわき/LConn2 -- _CN_132913106_500000_CN_104391636_500000/RConn2
  福島東幹線2_CN_106309481_500000_CN_104391636_500000/RConn3 -- T_104391636_500000_新いわき/LConn3 -- _CN_132913106_500000_CN_104391636_500000/RConn3
  G_103783431_福島第一_原子力発電所/RConn1 -- _CN_106309481_500000_CN103783431/RConn1
  G_103783431_福島第一_原子力発電所/RConn2 -- _CN_106309481_500000_CN103783431/RConn2
  G_103783431_福島第一_原子力発電所/RConn3 -- _CN_106309481_500000_CN103783431/RConn3
  T_190984572_275000_/LConn1 -- _CN_190984572_275000_CN191382966/LConn1
  T_190984572_275000_/LConn2 -- _CN_190984572_275000_CN191382966/LConn2
  T_190984572_275000_/LConn3 -- _CN_190984572_275000_CN191382966/LConn3
  G_191382966_喜撰山水力発電所/RConn1 -- _CN_190984572_275000_CN191382966/RConn1
  G_191382966_喜撰山水力発電所/RConn2 -- _CN_190984572_275000_CN191382966/RConn2
  G_191382966_喜撰山水力発電所/RConn3 -- _CN_190984572_275000_CN191382966/RConn3
  T_209726348_500000_信濃変電所/LConn1 -- 信濃幹線_CN_209726348_500000_CN_209429410_500000/LConn1
  T_209726348_500000_信濃変電所/LConn2 -- 信濃幹線_CN_209726348_500000_CN_209429410_500000/LConn2
  T_209726348_500000_信濃変電所/LConn3 -- 信濃幹線_CN_209726348_500000_CN_209429410_500000/LConn3
  信濃幹線_CN_209726348_500000_CN_209429410_500000/RConn1 -- T_209429410_500000_南信変電所/LConn1 -- 南信幹線_CN_209429410_500000_CN_142662111_500000/RConn1
  信濃幹線_CN_209726348_500000_CN_209429410_500000/RConn2 -- T_209429410_500000_南信変電所/LConn2 -- 南信幹線_CN_209429410_500000_CN_142662111_500000/RConn2
  信濃幹線_CN_209726348_500000_CN_209429410_500000/RConn3 -- T_209429410_500000_南信変電所/LConn3 -- 南信幹線_CN_209429410_500000_CN_142662111_500000/RConn3
  T_315662839_500000_新信濃変電所/LConn1 -- _CN_195615141_500000_CN_315662839_500000/RConn1
  T_315662839_500000_新信濃変電所/LConn2 -- _CN_195615141_500000_CN_315662839_500000/RConn2
  T_315662839_500000_新信濃変電所/LConn3 -- _CN_195615141_500000_CN_315662839_500000/RConn3
  T_109850439_500000_/LConn1 -- 阿南紀北直流幹線_CN_109850439_500000_CN_217885658_500000/LConn1
  T_109850439_500000_/LConn2 -- 阿南紀北直流幹線_CN_109850439_500000_CN_217885658_500000/LConn2
  T_109850439_500000_/LConn3 -- 阿南紀北直流幹線_CN_109850439_500000_CN_217885658_500000/LConn3
  阿南紀北直流幹線_CN_109850439_500000_CN_217885658_500000/RConn1 -- T_217885658_500000;0_由良開閉所/LConn1 -- L_217885658/LConn1
  阿南紀北直流幹線_CN_109850439_500000_CN_217885658_500000/RConn2 -- T_217885658_500000;0_由良開閉所/LConn2 -- L_217885658/LConn2
  阿南紀北直流幹線_CN_109850439_500000_CN_217885658_500000/RConn3 -- T_217885658_500000;0_由良開閉所/LConn3 -- L_217885658/LConn3
  G_233174201_/RConn1 -- _CN_232998815_275000_CN233174201/RConn1
  G_233174201_/RConn2 -- _CN_232998815_275000_CN233174201/RConn2
  G_233174201_/RConn3 -- _CN_232998815_275000_CN233174201/RConn3
  G_110340505_新神戸変電所/RConn1 -- _CN_185032690_275000_CN110340505/RConn1
  G_110340505_新神戸変電所/RConn2 -- _CN_185032690_275000_CN110340505/RConn2
  G_110340505_新神戸変電所/RConn3 -- _CN_185032690_275000_CN110340505/RConn3
  T_201293312_500000;220000_/RConn1 -- L_201293312/LConn1
  T_201293312_500000;220000_/RConn2 -- L_201293312/LConn2
  T_201293312_500000;220000_/RConn3 -- L_201293312/LConn3
  T_216778426_500000;220000_/RConn1 -- L_216778426/LConn1
  T_216778426_500000;220000_/RConn2 -- L_216778426/LConn2
  T_216778426_500000;220000_/RConn3 -- L_216778426/LConn3
  T_187988970_500000;220000_/RConn1 -- L_187988970/LConn1
  T_187988970_500000;220000_/RConn2 -- L_187988970/LConn2
  T_187988970_500000;220000_/RConn3 -- L_187988970/LConn3
  T_104173570_500000_/RConn1 -- L_104173570/LConn1
  T_104173570_500000_/RConn2 -- L_104173570/LConn2
  T_104173570_500000_/RConn3 -- L_104173570/LConn3
  T_106309481_500000_新福島変電所/RConn1 -- L_106309481/LConn1
  T_106309481_500000_新福島変電所/RConn2 -- L_106309481/LConn2
  T_106309481_500000_新福島変電所/RConn3 -- L_106309481/LConn3
  T_116828675_275000_北相模変電所_(Kita_Sagami_Hendensho)/RConn1 -- L_116828675/LConn1
  T_116828675_275000_北相模変電所_(Kita_Sagami_Hendensho)/RConn2 -- L_116828675/LConn2
  T_116828675_275000_北相模変電所_(Kita_Sagami_Hendensho)/RConn3 -- L_116828675/LConn3
  T_169121284_275000_/RConn1 -- L_169121284/LConn1
  T_169121284_275000_/RConn2 -- L_169121284/LConn2
  T_169121284_275000_/RConn3 -- L_169121284/LConn3
  T_169121278_275000_電源名古屋/RConn1 -- L_169121278/LConn1
  T_169121278_275000_電源名古屋/RConn2 -- L_169121278/LConn2
  T_169121278_275000_電源名古屋/RConn3 -- L_169121278/LConn3
  T_193544791_500000_新西広島変電所_(Shin_Nishi_Hiroshima_Hendensho)/RConn1 -- L_193544791/LConn1
  T_193544791_500000_新西広島変電所_(Shin_Nishi_Hiroshima_Hendensho)/RConn2 -- L_193544791/LConn2
  T_193544791_500000_新西広島変電所_(Shin_Nishi_Hiroshima_Hendensho)/RConn3 -- L_193544791/LConn3
  T_170974371_500000_新広島変電所_(Shin_Hiroshima_Hendensho)/RConn1 -- L_170974371/LConn1
  T_170974371_500000_新広島変電所_(Shin_Hiroshima_Hendensho)/RConn2 -- L_170974371/LConn2
  T_170974371_500000_新広島変電所_(Shin_Hiroshima_Hendensho)/RConn3 -- L_170974371/LConn3
  T_242253500_500000_東山口変電所_(Higashi_Yamaguchi_Hendensho)/RConn1 -- L_242253500/LConn1
  T_242253500_500000_東山口変電所_(Higashi_Yamaguchi_Hendensho)/RConn2 -- L_242253500/LConn2
  T_242253500_500000_東山口変電所_(Higashi_Yamaguchi_Hendensho)/RConn3 -- L_242253500/LConn3
  T_317416612_500000_西島根変電所/RConn1 -- L_317416612/LConn1
  T_317416612_500000_西島根変電所/RConn2 -- L_317416612/LConn2
  T_317416612_500000_西島根変電所/RConn3 -- L_317416612/LConn3
  T_161727149_500000_新生駒変電所_(Shin_Ikoma_Hendensho)/RConn1 -- L_161727149/LConn1
  T_161727149_500000_新生駒変電所_(Shin_Ikoma_Hendensho)/RConn2 -- L_161727149/LConn2
  T_161727149_500000_新生駒変電所_(Shin_Ikoma_Hendensho)/RConn3 -- L_161727149/LConn3
  T_169031921_500000_西京都変電所_(Nishi_Kyōto_Hendensho)/RConn1 -- L_169031921/LConn1
  T_169031921_500000_西京都変電所_(Nishi_Kyōto_Hendensho)/RConn2 -- L_169031921/LConn2
  T_169031921_500000_西京都変電所_(Nishi_Kyōto_Hendensho)/RConn3 -- L_169031921/LConn3
  T_169359724_500000_信貴変電所_(Shingi_Hendensho)/RConn1 -- L_169359724/LConn1
  T_169359724_500000_信貴変電所_(Shingi_Hendensho)/RConn2 -- L_169359724/LConn2
  T_169359724_500000_信貴変電所_(Shingi_Hendensho)/RConn3 -- L_169359724/LConn3
  T_161870227_500000_南京都変電所_(Minami_Kyōto_Hendensho)/RConn1 -- L_161870227/LConn1
  T_161870227_500000_南京都変電所_(Minami_Kyōto_Hendensho)/RConn2 -- L_161870227/LConn2
  T_161870227_500000_南京都変電所_(Minami_Kyōto_Hendensho)/RConn3 -- L_161870227/LConn3
  T_149843487_500000_新秦野変電所_(Shin_Hatano_Hendensho)/RConn1 -- L_149843487/LConn1
  T_149843487_500000_新秦野変電所_(Shin_Hatano_Hendensho)/RConn2 -- L_149843487/LConn2
  T_149843487_500000_新秦野変電所_(Shin_Hatano_Hendensho)/RConn3 -- L_149843487/LConn3
  T_150065045_500000_新富士変電所/RConn1 -- L_150065045/LConn1
  T_150065045_500000_新富士変電所/RConn2 -- L_150065045/LConn2
  T_150065045_500000_新富士変電所/RConn3 -- L_150065045/LConn3
  T_145079972_500000_新多摩変電所_(Shin_Tama_Substation)/RConn1 -- L_145079972/LConn1
  T_145079972_500000_新多摩変電所_(Shin_Tama_Substation)/RConn2 -- L_145079972/LConn2
  T_145079972_500000_新多摩変電所_(Shin_Tama_Substation)/RConn3 -- L_145079972/LConn3
  T_162844704_275000_中相模変電所/RConn1 -- L_162844704/LConn1
  T_162844704_275000_中相模変電所/RConn2 -- L_162844704/LConn2
  T_162844704_275000_中相模変電所/RConn3 -- L_162844704/LConn3
  T_128364781_275000_東京電力_京浜変電所/RConn1 -- L_128364781/LConn1
  T_128364781_275000_東京電力_京浜変電所/RConn2 -- L_128364781/LConn2
  T_128364781_275000_東京電力_京浜変電所/RConn3 -- L_128364781/LConn3
  T_150035494_500000_/RConn1 -- L_150035494/LConn1
  T_150035494_500000_/RConn2 -- L_150035494/LConn2
  T_150035494_500000_/RConn3 -- L_150035494/LConn3
  T_66098469_500000_西群馬開閉所/RConn1 -- L_66098469/LConn1
  T_66098469_500000_西群馬開閉所/RConn2 -- L_66098469/LConn2
  T_66098469_500000_西群馬開閉所/RConn3 -- L_66098469/LConn3
  T_170589736_500000_東近江/RConn1 -- L_170589736/LConn1
  T_170589736_500000_東近江/RConn2 -- L_170589736/LConn2
  T_170589736_500000_東近江/RConn3 -- L_170589736/LConn3
  T_170568495_500000_三重開閉所/RConn1 -- L_170568495/LConn1
  T_170568495_500000_三重開閉所/RConn2 -- L_170568495/LConn2
  T_170568495_500000_三重開閉所/RConn3 -- L_170568495/LConn3
  T_170537514_500000_/RConn1 -- L_170537514/LConn1
  T_170537514_500000_/RConn2 -- L_170537514/LConn2
  T_170537514_500000_/RConn3 -- L_170537514/LConn3
  T_192745005_275000_丸山変電所_(Maruyama_Hendensho)/RConn1 -- L_192745005/LConn1
  T_192745005_275000_丸山変電所_(Maruyama_Hendensho)/RConn2 -- L_192745005/LConn2
  T_192745005_275000_丸山変電所_(Maruyama_Hendensho)/RConn3 -- L_192745005/LConn3
  T_161946848_275000_関開閉所_(Seki)/RConn1 -- L_161946848/LConn1
  T_161946848_275000_関開閉所_(Seki)/RConn2 -- L_161946848/LConn2
  T_161946848_275000_関開閉所_(Seki)/RConn3 -- L_161946848/LConn3
  T_108199478_275000_南大阪変電所_(Minamiōsaka_Hendensho)/RConn1 -- L_108199478/LConn1
  T_108199478_275000_南大阪変電所_(Minamiōsaka_Hendensho)/RConn2 -- L_108199478/LConn2
  T_108199478_275000_南大阪変電所_(Minamiōsaka_Hendensho)/RConn3 -- L_108199478/LConn3
  T_109834508_275000_金剛開閉所_(Kongō_Kaiheisho)/RConn1 -- L_109834508/LConn1
  T_109834508_275000_金剛開閉所_(Kongō_Kaiheisho)/RConn2 -- L_109834508/LConn2
  T_109834508_275000_金剛開閉所_(Kongō_Kaiheisho)/RConn3 -- L_109834508/LConn3
  T_158522649_275000_東大阪変電所/RConn1 -- L_158522649/LConn1
  T_158522649_275000_東大阪変電所/RConn2 -- L_158522649/LConn2
  T_158522649_275000_東大阪変電所/RConn3 -- L_158522649/LConn3
  T_315614776_275000_/RConn1 -- L_315614776/LConn1
  T_315614776_275000_/RConn2 -- L_315614776/LConn2
  T_315614776_275000_/RConn3 -- L_315614776/LConn3
  T_315614783_275000_/RConn1 -- L_315614783/LConn1
  T_315614783_275000_/RConn2 -- L_315614783/LConn2
  T_315614783_275000_/RConn3 -- L_315614783/LConn3
  T_316566585_275000_/RConn1 -- L_316566585/LConn1
  T_316566585_275000_/RConn2 -- L_316566585/LConn2
  T_316566585_275000_/RConn3 -- L_316566585/LConn3
  T_174636874_275000_岩手変電所/RConn1 -- L_174636874/LConn1
  T_174636874_275000_岩手変電所/RConn2 -- L_174636874/LConn2
  T_174636874_275000_岩手変電所/RConn3 -- L_174636874/LConn3
  T_316566588_275000_/RConn1 -- L_316566588/LConn1
  T_316566588_275000_/RConn2 -- L_316566588/LConn2
  T_316566588_275000_/RConn3 -- L_316566588/LConn3
  T_316581632_275000_/RConn1 -- L_316581632/LConn1
  T_316581632_275000_/RConn2 -- L_316581632/LConn2
  T_316581632_275000_/RConn3 -- L_316581632/LConn3
  T_308348224_275000_新庄変電所/RConn1 -- L_308348224/LConn1
  T_308348224_275000_新庄変電所/RConn2 -- L_308348224/LConn2
  T_308348224_275000_新庄変電所/RConn3 -- L_308348224/LConn3
  T_116559939_500000_/RConn1 -- L_116559939/LConn1
  T_116559939_500000_/RConn2 -- L_116559939/LConn2
  T_116559939_500000_/RConn3 -- L_116559939/LConn3
  T_210090094_500000_駿遠変電所/RConn1 -- L_210090094/LConn1
  T_210090094_500000_駿遠変電所/RConn2 -- L_210090094/LConn2
  T_210090094_500000_駿遠変電所/RConn3 -- L_210090094/LConn3
  T_103818820_275000_仙台変電所/RConn1 -- L_103818820/LConn1
  T_103818820_275000_仙台変電所/RConn2 -- L_103818820/LConn2
  T_103818820_275000_仙台変電所/RConn3 -- L_103818820/LConn3
  T_318218831_275000_/RConn1 -- L_318218831/LConn1
  T_318218831_275000_/RConn2 -- L_318218831/LConn2
  T_318218831_275000_/RConn3 -- L_318218831/LConn3
  T_250430935_275000_米沢変電所_(Yonezawa_Hendensho)/RConn1 -- L_250430935/LConn1
  T_250430935_275000_米沢変電所_(Yonezawa_Hendensho)/RConn2 -- L_250430935/LConn2
  T_250430935_275000_米沢変電所_(Yonezawa_Hendensho)/RConn3 -- L_250430935/LConn3
  T_172601929_500000;220000_/RConn1 -- L_172601929/LConn1
  T_172601929_500000;220000_/RConn2 -- L_172601929/LConn2
  T_172601929_500000;220000_/RConn3 -- L_172601929/LConn3
  T_169993955_275000_新潟変電所/RConn1 -- L_169993955/LConn1
  T_169993955_275000_新潟変電所/RConn2 -- L_169993955/LConn2
  T_169993955_275000_新潟変電所/RConn3 -- L_169993955/LConn3
  T_319300956_275000_中越変電所/RConn1 -- L_319300956/LConn1
  T_319300956_275000_中越変電所/RConn2 -- L_319300956/LConn2
  T_319300956_275000_中越変電所/RConn3 -- L_319300956/LConn3
  T_170016148_275000_北新潟変電所/RConn1 -- L_170016148/LConn1
  T_170016148_275000_北新潟変電所/RConn2 -- L_170016148/LConn2
  T_170016148_275000_北新潟変電所/RConn3 -- L_170016148/LConn3
  T_158064651_275000_田子倉発電所/RConn1 -- L_158064651/LConn1
  T_158064651_275000_田子倉発電所/RConn2 -- L_158064651/LConn2
  T_158064651_275000_田子倉発電所/RConn3 -- L_158064651/LConn3
  T_232998815_275000_/RConn1 -- L_232998815/LConn1
  T_232998815_275000_/RConn2 -- L_232998815/LConn2
  T_232998815_275000_/RConn3 -- L_232998815/LConn3
